simulink model "ForwardKinematic_YuMi"  (R2024a)
(part 18 of 23)

(2579692110316253*sin(q1R))/4503599627370496))/36893488147419103232 + sin(q2R)*((2579692110316253*cos(q1R))/4503599627370496 - (1917820484151683*sin(q1R))/18014398509481984)))/36893488147419103232) + ((234819211581865*cos(q4R))/1152921504606846976 + (9007199067919185*sin(q4R))/9007199254740992)*((129801982932889585091297864435361917839115294955*cos(q1R))/5986310706507378352962293074805895248510699696029696 + (296957971066013582975066703729047659005068212725*cos(q2R))/365375409332725729550921208179070754913983135744 + (174598797980560374072834504815488878557302284405*sin(q1R))/1496577676626844588240573268701473812127674924007424 - (67682029681889335677290557259385*cos(q2R)*((1917820484151683*cos(q1R))/18014398509481984 + (2579692110316253*sin(q1R))/4503599627370496))/332306998946228968225951765070086144 + (9007199067919185*sin(q2R)*((2579692110316253*cos(q1R))/4503599627370496 - (1917820484151683*sin(q1R))/18014398509481984))/9007199254740992 + 206672498930123057048696703425560088887371380901/6129982163463555433433388108601236734474956488734408704)))/36893488147419103232 + sin(q5R)*(((7514214926474921*cos(q4R))/36893488147419103232 + (4503599440548691*sin(q4R))/4503599627370496)*(cos(q3R)*(cos(q2R)*((2579692110316253*cos(q1R))/4503599627370496 - (1917820484151683*sin(q1R))/18014398509481984) - (32968958366167862000829996477285*sin(q2R))/40564819207303340847894502572032 + (7514214926474921*sin(q2R)*((1917820484151683*cos(q1R))/18014398509481984 + (2579692110316253*sin(q1R))/4503599627370496))/36893488147419103232) - (9007199067919185*sin(q3R)*((17274190877287359225804725738355*cos(q1R))/162259276829213363391578010288128 + (23235800371559029388956996013805*sin(q1R))/40564819207303340847894502572032 + 27504203825998033884751021716381/166153499473114484112975882535043072))/9007199254740992 + (7514214926474921*sin(q3R)*((32968958366167862000829996477285*cos(q2R))/40564819207303340847894502572032 - (7514214926474921*cos(q2R)*((1917820484151683*cos(q1R))/18014398509481984 + (2579692110316253*sin(q1R))/4503599627370496))/36893488147419103232 + sin(q2R)*((2579692110316253*cos(q1R))/4503599627370496 - (1917820484151683*sin(q1R))/18014398509481984)))/36893488147419103232) - (7514214926474921*sin(q4R)*((9007199067919185*cos(q3R)*((17274190877287359225804725738355*cos(q1R))/162259276829213363391578010288128 + (23235800371559029388956996013805*sin(q1R))/40564819207303340847894502572032 + 27504203825998033884751021716381/166153499473114484112975882535043072))/9007199254740992 - (7514214926474921*cos(q3R)*((32968958366167862000829996477285*cos(q2R))/40564819207303340847894502572032 - (7514214926474921*cos(q2R)*((1917820484151683*cos(q1R))/18014398509481984 + (2579692110316253*sin(q1R))/4503599627370496))/36893488147419103232 + sin(q2R)*((2579692110316253*cos(q1R))/4503599627370496 - (1917820484151683*sin(q1R))/18014398509481984)))/36893488147419103232 + sin(q3R)*(cos(q2R)*((2579692110316253*cos(q1R))/4503599627370496 - (1917820484151683*sin(q1R))/18014398509481984) - (32968958366167862000829996477285*sin(q2R))/40564819207303340847894502572032 + (7514214926474921*sin(q2R)*((1917820484151683*cos(q1R))/18014398509481984 + (2579692110316253*sin(q1R))/4503599627370496))/36893488147419103232)))/36893488147419103232 + ((9007199067919185*cos(q4R))/9007199254740992 - (234819211581865*sin(q4R))/1152921504606846976)*((129801982932889585091297864435361917839115294955*cos(q1R))/5986310706507378352962293074805895248510699696029696 + (296957971066013582975066703729047659005068212725*cos(q2R))/365375409332725729550921208179070754913983135744 + (174598797980560374072834504815488878557302284405*sin(q1R))/1496577676626844588240573268701473812127674924007424 - (67682029681889335677290557259385*cos(q2R)*((1917820484151683*cos(q1R))/18014398509481984 + (2579692110316253*sin(q1R))/4503599627370496))/332306998946228968225951765070086144 + (9007199067919185*sin(q2R)*((2579692110316253*cos(q1R))/4503599627370496 - (1917820484151683*sin(q1R))/18014398509481984))/9007199254740992 + 206672498930123057048696703425560088887371380901/6129982163463555433433388108601236734474956488734408704))))/9007199254740992000, (584133382113593486367040631332731*sin(q6R)*((1528559695827542654859482295756575375660057523072748460051910118126597762297125*cos(q1R))/8343699359066055009355553539724812947666814540455674882605631280555545803830627148527195652096 + (3497003479222003021661409533057350838749300515155764632398442290070889008826875*cos(q2R))/509258994083621521567111422102344540262867098416484062659035112338595324940834176545849344 + (2056090974134078155817856050893176283501835309672875224633265471054954772650875*sin(q1R))/2085924839766513752338888384931203236916703635113918720651407820138886450957656787131798913024 - (609625514665592237562888769449172969868262801225*cos(q3R)*((17274190877287359225804725738355*cos(q1R))/162259276829213363391578010288128 + (23235800371559029388956996013805*sin(q1R))/40564819207303340847894502572032 + 27504203825998033884751021716381/166153499473114484112975882535043072))/2993155353253689176481146537402947624255349848014848 + (15893040848161638993908057577265778144967053025*sin(q3R)*((17274190877287359225804725738355*cos(q1R))/162259276829213363391578010288128 + (23235800371559029388956996013805*sin(q1R))/40564819207303340847894502572032 + 27504203825998033884751021716381/166153499473114484112975882535043072))/383123885216472214589586756787577295904684780545900544 - (9007199067919185*((4503599440548691*cos(q4R))/4503599627370496 - (7514214926474921*sin(q4R))/36893488147419103232)*(cos(q3R)*(cos(q2R)*((2579692110316253*cos(q1R))/4503599627370496 - (1917820484151683*sin(q1R))/18014398509481984) - (32968958366167862000829996477285*sin(q2R))/40564819207303340847894502572032 + (7514214926474921*sin(q2R)*((1917820484151683*cos(q1R))/18014398509481984 + (2579692110316253*sin(q1R))/4503599627370496))/36893488147419103232) - (9007199067919185*sin(q3R)*((17274190877287359225804725738355*cos(q1R))/162259276829213363391578010288128 + (23235800371559029388956996013805*sin(q1R))/40564819207303340847894502572032 + 27504203825998033884751021716381/166153499473114484112975882535043072))/9007199254740992 + (7514214926474921*sin(q3R)*((32968958366167862000829996477285*cos(q2R))/40564819207303340847894502572032 - (7514214926474921*cos(q2R)*((1917820484151683*cos(q1R))/18014398509481984 + (2579692110316253*sin(q1R))/4503599627370496))/36893488147419103232 + sin(q2R)*((2579692110316253*cos(q1R))/4503599627370496 - (1917820484151683*sin(q1R))/18014398509481984)))/36893488147419103232))/9007199254740992 + (508577317689771495245073589786522929324694383585*cos(q3R)*((32968958366167862000829996477285*cos(q2R))/40564819207303340847894502572032 - (7514214926474921*cos(q2R)*((1917820484151683*cos(q1R))/18014398509481984 + (2579692110316253*sin(q1R))/4503599627370496))/36893488147419103232 + sin(q2R)*((2579692110316253*cos(q1R))/4503599627370496 - (1917820484151683*sin(q1R))/18014398509481984)))/12259964326927110866866776217202473468949912977468817408 - (1764482024691522628700660907665*cos(q3R)*(cos(q2R)*((2579692110316253*cos(q1R))/4503599627370496 - (1917820484151683*sin(q1R))/18014398509481984) - (32968958366167862000829996477285*sin(q2R))/40564819207303340847894502572032 + (7514214926474921*sin(q2R)*((1917820484151683*cos(q1R))/18014398509481984 + (2579692110316253*sin(q1R))/4503599627370496))/36893488147419103232))/42535295865117307932921825928971026432 - (13258697167433729449897784796786197386719169465*sin(q3R)*((32968958366167862000829996477285*cos(q2R))/40564819207303340847894502572032 - (7514214926474921*cos(q2R)*((1917820484151683*cos(q1R))/18014398509481984 + (2579692110316253*sin(q1R))/4503599627370496))/36893488147419103232 + sin(q2R)*((2579692110316253*cos(q1R))/4503599627370496 - (1917820484151683*sin(q1R))/18014398509481984)))/1569275433846670190958947355801916604025588861116008628224 - (67682029681889335677290557259385*sin(q3R)*(cos(q2R)*((2579692110316253*cos(q1R))/4503599627370496 - (1917820484151683*sin(q1R))/18014398509481984) - (32968958366167862000829996477285*sin(q2R))/40564819207303340847894502572032 + (7514214926474921*sin(q2R)*((1917820484151683*cos(q1R))/18014398509481984 + (2579692110316253*sin(q1R))/4503599627370496))/36893488147419103232))/332306998946228968225951765070086144 + (67682029681889335677290557259385*cos(q4R)*((9007199067919185*cos(q3R)*((17274190877287359225804725738355*cos(q1R))/162259276829213363391578010288128 + (23235800371559029388956996013805*sin(q1R))/40564819207303340847894502572032 + 27504203825998033884751021716381/166153499473114484112975882535043072))/9007199254740992 - (7514214926474921*cos(q3R)*((32968958366167862000829996477285*cos(q2R))/40564819207303340847894502572032 - (7514214926474921*cos(q2R)*((1917820484151683*cos(q1R))/18014398509481984 + (2579692110316253*sin(q1R))/4503599627370496))/36893488147419103232 + sin(q2R)*((2579692110316253*cos(q1R))/4503599627370496 - (1917820484151683*sin(q1R))/18014398509481984)))/36893488147419103232 + sin(q3R)*(cos(q2R)*((2579692110316253*cos(q1R))/4503599627370496 - (1917820484151683*sin(q1R))/18014398509481984) - (32968958366167862000829996477285*sin(q2R))/40564819207303340847894502572032 + (7514214926474921*sin(q2R)*((1917820484151683*cos(q1R))/18014398509481984 + (2579692110316253*sin(q1R))/4503599627370496))/36893488147419103232)))/332306998946228968225951765070086144 + (9007199067919185*((234819211581865*cos(q4R))/1152921504606846976 + (9007199067919185*sin(q4R))/9007199254740992)*((129801982932889585091297864435361917839115294955*cos(q1R))/5986310706507378352962293074805895248510699696029696 + (296957971066013582975066703729047659005068212725*cos(q2R))/365375409332725729550921208179070754913983135744 + (174598797980560374072834504815488878557302284405*sin(q1R))/1496577676626844588240573268701473812127674924007424 - (67682029681889335677290557259385*cos(q2R)*((1917820484151683*cos(q1R))/18014398509481984 + (2579692110316253*sin(q1R))/4503599627370496))/332306998946228968225951765070086144 + (9007199067919185*sin(q2R)*((2579692110316253*cos(q1R))/4503599627370496 - (1917820484151683*sin(q1R))/18014398509481984))/9007199254740992 + 206672498930123057048696703425560088887371380901/6129982163463555433433388108601236734474956488734408704))/9007199254740992 - (797029601289130257223357069404502671534492977261568326111352375*cos(q2R)*((1917820484151683*cos(q1R))/18014398509481984 + (2579692110316253*sin(q1R))/4503599627370496))/463168356949264781694283940034751631413079938662562256157830336031652518559744 + (106069577339469832923929692356850887620017617375*sin(q2R)*((2579692110316253*cos(q1R))/4503599627370496 - (1917820484151683*sin(q1R))/18014398509481984))/12554203470773361527671578846415332832204710888928069025792 + 2433793729205816076131138531933890152433695130941136279164373721607455952153675/8543948143683640329580086824678208458410818089426611079788166431288878903122562200091848347746304))/16225927682921336339157801028812800 - (48638874966763599*cos(q6R)*((1528559695827542654859482295756575375660057523072748460051910118126597762297125*cos(q1R))/8343699359066055009355553539724812947666814540455674882605631280555545803830627148527195652096 + (3497003479222003021661409533057350838749300515155764632398442290070889008826875*cos(q2R))/509258994083621521567111422102344540262867098416484062659035112338595324940834176545849344 + (2056090974134078155817856050893176283501835309672875224633265471054954772650875*sin(q1R))/2085924839766513752338888384931203236916703635113918720651407820138886450957656787131798913024 - (609625514665592237562888769449172969868262801225*cos(q3R)*((17274190877287359225804725738355*cos(q1R))/162259276829213363391578010288128 + (23235800371559029388956996013805*sin(q1R))/40564819207303340847894502572032 + 27504203825998033884751021716381/166153499473114484112975882535043072))/2993155353253689176481146537402947624255349848014848 + (15893040848161638993908057577265778144967053025*sin(q3R)*((17274190877287359225804725738355*cos(q1R))/162259276829213363391578010288128 + (23235800371559029388956996013805*sin(q1R))/40564819207303340847894502572032 + 27504203825998033884751021716381/166153499473114484112975882535043072))/383123885216472214589586756787577295904684780545900544 - (9007199067919185*((4503599440548691*cos(q4R))/4503599627370496 - (7514214926474921*sin(q4R))/36893488147419103232)*(cos(q3R)*(cos(q2R)*((2579692110316253*cos(q1R))/4503599627370496 - (1917820484151683*sin(q1R))/18014398509481984) - (32968958366167862000829996477285*sin(q2R))/40564819207303340847894502572032 + (7514214926474921*sin(q2R)*((1917820484151683*cos(q1R))/18014398509481984 + (2579692110316253*sin(q1R))/4503599627370496))/36893488147419103232) - (9007199067919185*sin(q3R)*((17274190877287359225804725738355*cos(q1R))/162259276829213363391578010288128 + (23235800371559029388956996013805*sin(q1R))/40564819207303340847894502572032 + 27504203825998033884751021716381/166153499473114484112975882535043072))/9007199254740992 + (7514214926474921*sin(q3R)*((32968958366167862000829996477285*cos(q2R))/40564819207303340847894502572032 - (7514214926474921*cos(q2R)*((1917820484151683*cos(q1R))/18014398509481984 + (2579692110316253*sin(q1R))/4503599627370496))/36893488147419103232 + sin(q2R)*((2579692110316253*cos(q1R))/4503599627370496 - (1917820484151683*sin(q1R))/18014398509481984)))/36893488147419103232))/9007199254740992 + (508577317689771495245073589786522929324694383585*cos(q3R)*((32968958366167862000829996477285*cos(q2R))/40564819207303340847894502572032 - (7514214926474921*cos(q2R)*((1917820484151683*cos(q1R))/18014398509481984 + (2579692110316253*sin(q1R))/4503599627370496))/36893488147419103232 + sin(q2R)*((2579692110316253*cos(q1R))/4503599627370496 - (1917820484151683*sin(q1R))/18014398509481984)))/12259964326927110866866776217202473468949912977468817408 - (1764482024691522628700660907665*cos(q3R)*(cos(q2R)*((2579692110316253*cos(q1R))/4503599627370496 - (1917820484151683*sin(q1R))/18014398509481984) - (32968958366167862000829996477285*sin(q2R))/40564819207303340847894502572032 + (7514214926474921*sin(q2R)*((1917820484151683*cos(q1R))/18014398509481984 + (2579692110316253*sin(q1R))/4503599627370496))/36893488147419103232))/42535295865117307932921825928971026432 - (13258697167433729449897784796786197386719169465*sin(q3R)*((32968958366167862000829996477285*cos(q2R))/40564819207303340847894502572032 - (7514214926474921*cos(q2R)*((1917820484151683*cos(q1R))/18014398509481984 + (2579692110316253*sin(q1R))/4503599627370496))/36893488147419103232 + sin(q2R)*((2579692110316253*cos(q1R))/4503599627370496 - (1917820484151683*sin(q1R))/18014398509481984)))/1569275433846670190958947355801916604025588861116008628224 - (67682029681889335677290557259385*sin(q3R)*(cos(q2R)*((2579692110316253*cos(q1R))/4503599627370496 - (1917820484151683*sin(q1R))/18014398509481984) - (32968958366167862000829996477285*sin(q2R))/40564819207303340847894502572032 + (7514214926474921*sin(q2R)*((1917820484151683*cos(q1R))/18014398509481984 + (2579692110316253*sin(q1R))/4503599627370496))/36893488147419103232))/332306998946228968225951765070086144 + (67682029681889335677290557259385*cos(q4R)*((9007199067919185*cos(q3R)*((17274190877287359225804725738355*cos(q1R))/162259276829213363391578010288128 + (23235800371559029388956996013805*sin(q1R))/40564819207303340847894502572032 + 27504203825998033884751021716381/166153499473114484112975882535043072))/9007199254740992 - (7514214926474921*cos(q3R)*((32968958366167862000829996477285*cos(q2R))/40564819207303340847894502572032 - (7514214926474921*cos(q2R)*((1917820484151683*cos(q1R))/18014398509481984 + (2579692110316253*sin(q1R))/4503599627370496))/36893488147419103232 + sin(q2R)*((2579692110316253*cos(q1R))/4503599627370496 - (1917820484151683*sin(q1R))/18014398509481984)))/36893488147419103232 + sin(q3R)*(cos(q2R)*((2579692110316253*cos(q1R))/4503599627370496 - (1917820484151683*sin(q1R))/18014398509481984) - (32968958366167862000829996477285*sin(q2R))/40564819207303340847894502572032 + (7514214926474921*sin(q2R)*((1917820484151683*cos(q1R))/18014398509481984 + (2579692110316253*sin(q1R))/4503599627370496))/36893488147419103232)))/332306998946228968225951765070086144 + (9007199067919185*((234819211581865*cos(q4R))/1152921504606846976 + (9007199067919185*sin(q4R))/9007199254740992)*((129801982932889585091297864435361917839115294955*cos(q1R))/5986310706507378352962293074805895248510699696029696 + (296957971066013582975066703729047659005068212725*cos(q2R))/365375409332725729550921208179070754913983135744 + (174598797980560374072834504815488878557302284405*sin(q1R))/1496577676626844588240573268701473812127674924007424 - (67682029681889335677290557259385*cos(q2R)*((1917820484151683*cos(q1R))/18014398509481984 + (2579692110316253*sin(q1R))/4503599627370496))/332306998946228968225951765070086144 + (9007199067919185*sin(q2R)*((2579692110316253*cos(q1R))/4503599627370496 - (1917820484151683*sin(q1R))/18014398509481984))/9007199254740992 + 206672498930123057048696703425560088887371380901/6129982163463555433433388108601236734474956488734408704))/9007199254740992 - (797029601289130257223357069404502671534492977261568326111352375*cos(q2R)*((1917820484151683*cos(q1R))/18014398509481984 + (2579692110316253*sin(q1R))/4503599627370496))/463168356949264781694283940034751631413079938662562256157830336031652518559744 + (106069577339469832923929692356850887620017617375*sin(q2R)*((2579692110316253*cos(q1R))/4503599627370496 - (1917820484151683*sin(q1R))/18014398509481984))/12554203470773361527671578846415332832204710888928069025792 + 2433793729205816076131138531933890152433695130941136279164373721607455952153675/8543948143683640329580086824678208458410818089426611079788166431288878903122562200091848347746304))/1801439850948198400 - (27*sin(q6R)*(cos(q5R)*(((7514214926474921*cos(q4R))/36893488147419103232 + (4503599440548691*sin(q4R))/4503599627370496)*(cos(q3R)*(cos(q2R)*((2579692110316253*cos(q1R))/4503599627370496 - (1917820484151683*sin(q1R))/18014398509481984) - (32968958366167862000829996477285*sin(q2R))/40564819207303340847894502572032 + (7514214926474921*sin(q2R)*((1917820484151683*cos(q1R))/18014398509481984 + (2579692110316253*sin(q1R))/4503599627370496))/36893488147419103232) - (9007199067919185*sin(q3R)*((17274190877287359225804725738355*cos(q1R))/162259276829213363391578010288128 + (23235800371559029388956996013805*sin(q1R))/40564819207303340847894502572032 + 27504203825998033884751021716381/166153499473114484112975882535043072))/9007199254740992 + (7514214926474921*sin(q3R)*((32968958366167862000829996477285*cos(q2R))/40564819207303340847894502572032 - (7514214926474921*cos(q2R)*((1917820484151683*cos(q1R))/18014398509481984 + (2579692110316253*sin(q1R))/4503599627370496))/36893488147419103232 + sin(q2R)*((2579692110316253*cos(q1R))/4503599627370496 - (1917820484151683*sin(q1R))/18014398509481984)))/36893488147419103232) - (7514214926474921*sin(q4R)*((9007199067919185*cos(q3R)*((17274190877287359225804725738355*cos(q1R))/162259276829213363391578010288128 + (23235800371559029388956996013805*sin(q1R))/40564819207303340847894502572032 + 27504203825998033884751021716381/166153499473114484112975882535043072))/9007199254740992 - (7514214926474921*cos(q3R)*((32968958366167862000829996477285*cos(q2R))/40564819207303340847894502572032 - (7514214926474921*cos(q2R)*((1917820484151683*cos(q1R))/18014398509481984 + (2579692110316253*sin(q1R))/4503599627370496))/36893488147419103232 + sin(q2R)*((2579692110316253*cos(q1R))/4503599627370496 - (1917820484151683*sin(q1R))/18014398509481984)))/36893488147419103232 + sin(q3R)*(cos(q2R)*((2579692110316253*cos(q1R))/4503599627370496 - (1917820484151683*sin(q1R))/18014398509481984) - (32968958366167862000829996477285*sin(q2R))/40564819207303340847894502572032 + (7514214926474921*sin(q2R)*((1917820484151683*cos(q1R))/18014398509481984 + (2579692110316253*sin(q1R))/4503599627370496))/36893488147419103232)))/36893488147419103232 + ((9007199067919185*cos(q4R))/9007199254740992 - (234819211581865*sin(q4R))/1152921504606846976)*((129801982932889585091297864435361917839115294955*cos(q1R))/5986310706507378352962293074805895248510699696029696 + (296957971066013582975066703729047659005068212725*cos(q2R))/365375409332725729550921208179070754913983135744 + (174598797980560374072834504815488878557302284405*sin(q1R))/1496577676626844588240573268701473812127674924007424 - (67682029681889335677290557259385*cos(q2R)*((1917820484151683*cos(q1R))/18014398509481984 + (2579692110316253*sin(q1R))/4503599627370496))/332306998946228968225951765070086144 + (9007199067919185*sin(q2R)*((2579692110316253*cos(q1R))/4503599627370496 - (1917820484151683*sin(q1R))/18014398509481984))/9007199254740992 + 206672498930123057048696703425560088887371380901/6129982163463555433433388108601236734474956488734408704)) - (9007199067919185*sin(q5R)*((203422408166946418981152780445187297537016008229516441756292125*cos(q1R))/226156424291633194186662080095093570025917938800079226639565593765455331328 + (465385075279251052437186083221547446448384963368966483726351875*cos(q2R))/13803492693581127574869511724554050904902217944340773110325048447598592 + (273626851807209941619219010639387076236787289365779842797695875*sin(q1R))/56539106072908298546665520023773392506479484700019806659891398441363832832 - (81129635049124235038645691064225*cos(q3R)*((17274190877287359225804725738355*cos(q1R))/162259276829213363391578010288128 + (23235800371559029388956996013805*sin(q1R))/40564819207303340847894502572032 + 27504203825998033884751021716381/166153499473114484112975882535043072))/81129638414606681695789005144064 + (2115063383689692319117831580025*sin(q3R)*((17274190877287359225804725738355*cos(q1R))/162259276829213363391578010288128 + (23235800371559029388956996013805*sin(q1R))/40564819207303340847894502572032 + 27504203825998033884751021716381/166153499473114484112975882535043072))/10384593717069655257060992658440192 + (67682029681889335677290557259385*cos(q3R)*((32968958366167862000829996477285*cos(q2R))/40564819207303340847894502572032 - (7514214926474921*cos(q2R)*((1917820484151683*cos(q1R))/18014398509481984 + (2579692110316253*sin(q1R))/4503599627370496))/36893488147419103232 + sin(q2R)*((2579692110316253*cos(q1R))/4503599627370496 - (1917820484151683*sin(q1R))/18014398509481984)))/332306998946228968225951765070086144 - (234819211581865*cos(q3R)*(cos(q2R)*((2579692110316253*cos(q1R))/4503599627370496 - (1917820484151683*sin(q1R))/18014398509481984) - (32968958366167862000829996477285*sin(q2R))/40564819207303340847894502572032 + (7514214926474921*sin(q2R)*((1917820484151683*cos(q1R))/18014398509481984 + (2579692110316253*sin(q1R))/4503599627370496))/36893488147419103232))/1152921504606846976 - (1764482024691522628700660907665*sin(q3R)*((32968958366167862000829996477285*cos(q2R))/40564819207303340847894502572032 - (7514214926474921*cos(q2R)*((1917820484151683*cos(q1R))/18014398509481984 + (2579692110316253*sin(q1R))/4503599627370496))/36893488147419103232 + sin(q2R)*((2579692110316253*cos(q1R))/4503599627370496 - (1917820484151683*sin(q1R))/18014398509481984)))/42535295865117307932921825928971026432 - (9007199067919185*sin(q3R)*(cos(q2R)*((2579692110316253*cos(q1R))/4503599627370496 - (1917820484151683*sin(q1R))/18014398509481984) - (32968958366167862000829996477285*sin(q2R))/40564819207303340847894502572032 + (7514214926474921*sin(q2R)*((1917820484151683*cos(q1R))/18014398509481984 + (2579692110316253*sin(q1R))/4503599627370496))/36893488147419103232))/9007199254740992 - (106069577339469832923929692356850887620017617375*cos(q2R)*((1917820484151683*cos(q1R))/18014398509481984 + (2579692110316253*sin(q1R))/4503599627370496))/12554203470773361527671578846415332832204710888928069025792 + (14115856197532180673579726082375*sin(q2R)*((2579692110316253*cos(q1R))/4503599627370496 - (1917820484151683*sin(q1R))/18014398509481984))/340282366920938463463374607431768211456 + 323891950525769801103968238055131782751500431270071838086942675/231584178474632390847141970017375815706539969331281128078915168015826259279872))/9007199254740992 + (7514214926474921*sin(q5R)*((7514214926474921*cos(q4R)*((9007199067919185*cos(q3R)*((17274190877287359225804725738355*cos(q1R))/162259276829213363391578010288128 + (23235800371559029388956996013805*sin(q1R))/40564819207303340847894502572032 + 27504203825998033884751021716381/166153499473114484112975882535043072))/9007199254740992 - (7514214926474921*cos(q3R)*((32968958366167862000829996477285*cos(q2R))/40564819207303340847894502572032 - (7514214926474921*cos(q2R)*((1917820484151683*cos(q1R))/18014398509481984 + (2579692110316253*sin(q1R))/4503599627370496))/36893488147419103232 + sin(q2R)*((2579692110316253*cos(q1R))/4503599627370496 - (1917820484151683*sin(q1R))/18014398509481984)))/36893488147419103232 + sin(q3R)*(cos(q2R)*((2579692110316253*cos(q1R))/4503599627370496 - (1917820484151683*sin(q1R))/18014398509481984) - (32968958366167862000829996477285*sin(q2R))/40564819207303340847894502572032 + (7514214926474921*sin(q2R)*((1917820484151683*cos(q1R))/18014398509481984 + (2579692110316253*sin(q1R))/4503599627370496))/36893488147419103232)))/36893488147419103232 - ((4503599440548691*cos(q4R))/4503599627370496 - (7514214926474921*sin(q4R))/36893488147419103232)*(cos(q3R)*(cos(q2R)*((2579692110316253*cos(q1R))/4503599627370496 - (1917820484151683*sin(q1R))/18014398509481984) - (32968958366167862000829996477285*sin(q2R))/40564819207303340847894502572032 + (7514214926474921*sin(q2R)*((1917820484151683*cos(q1R))/18014398509481984 + (2579692110316253*sin(q1R))/4503599627370496))/36893488147419103232) - (9007199067919185*sin(q3R)*((17274190877287359225804725738355*cos(q1R))/162259276829213363391578010288128 + (23235800371559029388956996013805*sin(q1R))/40564819207303340847894502572032 + 27504203825998033884751021716381/166153499473114484112975882535043072))/9007199254740992 + (7514214926474921*sin(q3R)*((32968958366167862000829996477285*cos(q2R))/40564819207303340847894502572032 - (7514214926474921*cos(q2R)*((1917820484151683*cos(q1R))/18014398509481984 + (2579692110316253*sin(q1R))/4503599627370496))/36893488147419103232 + sin(q2R)*((2579692110316253*cos(q1R))/4503599627370496 - (1917820484151683*sin(q1R))/18014398509481984)))/36893488147419103232) + ((234819211581865*cos(q4R))/1152921504606846976 + (9007199067919185*sin(q4R))/9007199254740992)*((129801982932889585091297864435361917839115294955*cos(q1R))/5986310706507378352962293074805895248510699696029696 + (296957971066013582975066703729047659005068212725*cos(q2R))/365375409332725729550921208179070754913983135744 + (174598797980560374072834504815488878557302284405*sin(q1R))/1496577676626844588240573268701473812127674924007424 - (67682029681889335677290557259385*cos(q2R)*((1917820484151683*cos(q1R))/18014398509481984 + (2579692110316253*sin(q1R))/4503599627370496))/332306998946228968225951765070086144 + (9007199067919185*sin(q2R)*((2579692110316253*cos(q1R))/4503599627370496 - (1917820484151683*sin(q1R))/18014398509481984))/9007199254740992 + 206672498930123057048696703425560088887371380901/6129982163463555433433388108601236734474956488734408704)))/36893488147419103232))/1000 + (202883803014822867*cos(q6R)*((9007199067919185*cos(q5R)*((203422408166946418981152780445187297537016008229516441756292125*cos(q1R))/226156424291633194186662080095093570025917938800079226639565593765455331328 + (465385075279251052437186083221547446448384963368966483726351875*cos(q2R))/13803492693581127574869511724554050904902217944340773110325048447598592 + (273626851807209941619219010639387076236787289365779842797695875*sin(q1R))/56539106072908298546665520023773392506479484700019806659891398441363832832 - (81129635049124235038645691064225*cos(q3R)*((17274190877287359225804725738355*cos(q1R))/162259276829213363391578010288128 + (23235800371559029388956996013805*sin(q1R))/40564819207303340847894502572032 + 27504203825998033884751021716381/166153499473114484112975882535043072))/81129638414606681695789005144064 + (2115063383689692319117831580025*sin(q3R)*((17274190877287359225804725738355*cos(q1R))/162259276829213363391578010288128 + (23235800371559029388956996013805*sin(q1R))/40564819207303340847894502572032 + 27504203825998033884751021716381/166153499473114484112975882535043072))/10384593717069655257060992658440192 + (67682029681889335677290557259385*cos(q3R)*((32968958366167862000829996477285*cos(q2R))/40564819207303340847894502572032 - (7514214926474921*cos(q2R)*((1917820484151683*cos(q1R))/18014398509481984 + (2579692110316253*sin(q1R))/4503599627370496))/36893488147419103232 + sin(q2R)*((2579692110316253*cos(q1R))/4503599627370496 - (1917820484151683*sin(q1R))/18014398509481984)))/332306998946228968225951765070086144 - (234819211581865*cos(q3R)*(cos(q2R)*((2579692110316253*cos(q1R))/4503599627370496 - (1917820484151683*sin(q1R))/18014398509481984) - (32968958366167862000829996477285*sin(q2R))/40564819207303340847894502572032 + (7514214926474921*sin(q2R)*((1917820484151683*cos(q1R))/18014398509481984 + (2579692110316253*sin(q1R))/4503599627370496))/36893488147419103232))/1152921504606846976 - (1764482024691522628700660907665*sin(q3R)*((32968958366167862000829996477285*cos(q2R))/40564819207303340847894502572032 - (7514214926474921*cos(q2R)*((1917820484151683*cos(q1R))/18014398509481984 + (2579692110316253*sin(q1R))/4503599627370496))/36893488147419103232 + sin(q2R)*((2579692110316253*cos(q1R))/4503599627370496 - (1917820484151683*sin(q1R))/18014398509481984)))/42535295865117307932921825928971026432 - (9007199067919185*sin(q3R)*(cos(q2R)*((2579692110316253*cos(q1R))/4503599627370496 - (1917820484151683*sin(q1R))/18014398509481984) - (32968958366167862000829996477285*sin(q2R))/40564819207303340847894502572032 + (7514214926474921*sin(q2R)*((1917820484151683*cos(q1R))/18014398509481984 + (2579692110316253*sin(q1R))/4503599627370496))/36893488147419103232))/9007199254740992 - (106069577339469832923929692356850887620017617375*cos(q2R)*((1917820484151683*cos(q1R))/18014398509481984 + (2579692110316253*sin(q1R))/4503599627370496))/12554203470773361527671578846415332832204710888928069025792 + (14115856197532180673579726082375*sin(q2R)*((2579692110316253*cos(q1R))/4503599627370496 - (1917820484151683*sin(q1R))/18014398509481984))/340282366920938463463374607431768211456 + 323891950525769801103968238055131782751500431270071838086942675/231584178474632390847141970017375815706539969331281128078915168015826259279872))/9007199254740992 - (7514214926474921*cos(q5R)*((7514214926474921*cos(q4R)*((9007199067919185*cos(q3R)*((17274190877287359225804725738355*cos(q1R))/162259276829213363391578010288128 + (23235800371559029388956996013805*sin(q1R))/40564819207303340847894502572032 + 27504203825998033884751021716381/166153499473114484112975882535043072))/9007199254740992 - (7514214926474921*cos(q3R)*((32968958366167862000829996477285*cos(q2R))/40564819207303340847894502572032 - (7514214926474921*cos(q2R)*((1917820484151683*cos(q1R))/18014398509481984 + (2579692110316253*sin(q1R))/4503599627370496))/36893488147419103232 + sin(q2R)*((2579692110316253*cos(q1R))/4503599627370496 - (1917820484151683*sin(q1R))/18014398509481984)))/36893488147419103232 + sin(q3R)*(cos(q2R)*((2579692110316253*cos(q1R))/4503599627370496 - (1917820484151683*sin(q1R))/18014398509481984) - (32968958366167862000829996477285*sin(q2R))/40564819207303340847894502572032 + (7514214926474921*sin(q2R)*((1917820484151683*cos(q1R))/18014398509481984 + (2579692110316253*sin(q1R))/4503599627370496))/36893488147419103232)))/36893488147419103232 - ((4503599440548691*cos(q4R))/4503599627370496 - (7514214926474921*sin(q4R))/36893488147419103232)*(cos(q3R)*(cos(q2R)*((2579692110316253*cos(q1R))/4503599627370496 - (1917820484151683*sin(q1R))/18014398509481984) - (32968958366167862000829996477285*sin(q2R))/40564819207303340847894502572032 + (7514214926474921*sin(q2R)*((1917820484151683*cos(q1R))/18014398509481984 + (2579692110316253*sin(q1R))/4503599627370496))/36893488147419103232) - (9007199067919185*sin(q3R)*((17274190877287359225804725738355*cos(q1R))/162259276829213363391578010288128 + (23235800371559029388956996013805*sin(q1R))/40564819207303340847894502572032 + 27504203825998033884751021716381/166153499473114484112975882535043072))/9007199254740992 + (7514214926474921*sin(q3R)*((32968958366167862000829996477285*cos(q2R))/40564819207303340847894502572032 - (7514214926474921*cos(q2R)*((1917820484151683*cos(q1R))/18014398509481984 + (2579692110316253*sin(q1R))/4503599627370496))/36893488147419103232 + sin(q2R)*((2579692110316253*cos(q1R))/4503599627370496 - (1917820484151683*sin(q1R))/18014398509481984)))/36893488147419103232) + ((234819211581865*cos(q4R))/1152921504606846976 + (9007199067919185*sin(q4R))/9007199254740992)*((129801982932889585091297864435361917839115294955*cos(q1R))/5986310706507378352962293074805895248510699696029696 + (296957971066013582975066703729047659005068212725*cos(q2R))/365375409332725729550921208179070754913983135744 + (174598797980560374072834504815488878557302284405*sin(q1R))/1496577676626844588240573268701473812127674924007424 - (67682029681889335677290557259385*cos(q2R)*((1917820484151683*cos(q1R))/18014398509481984 + (2579692110316253*sin(q1R))/4503599627370496))/332306998946228968225951765070086144 + (9007199067919185*sin(q2R)*((2579692110316253*cos(q1R))/4503599627370496 - (1917820484151683*sin(q1R))/18014398509481984))/9007199254740992 + 206672498930123057048696703425560088887371380901/6129982163463555433433388108601236734474956488734408704)))/36893488147419103232 + sin(q5R)*(((7514214926474921*cos(q4R))/36893488147419103232 + (4503599440548691*sin(q4R))/4503599627370496)*(cos(q3R)*(cos(q2R)*((2579692110316253*cos(q1R))/4503599627370496 - (1917820484151683*sin(q1R))/18014398509481984) - (32968958366167862000829996477285*sin(q2R))/40564819207303340847894502572032 + (7514214926474921*sin(q2R)*((1917820484151683*cos(q1R))/18014398509481984 + (2579692110316253*sin(q1R))/4503599627370496))/36893488147419103232) - (9007199067919185*sin(q3R)*((17274190877287359225804725738355*cos(q1R))/162259276829213363391578010288128 + (23235800371559029388956996013805*sin(q1R))/40564819207303340847894502572032 + 27504203825998033884751021716381/166153499473114484112975882535043072))/9007199254740992 + (7514214926474921*sin(q3R)*((32968958366167862000829996477285*cos(q2R))/40564819207303340847894502572032 - (7514214926474921*cos(q2R)*((1917820484151683*cos(q1R))/18014398509481984 + (2579692110316253*sin(q1R))/4503599627370496))/36893488147419103232 + sin(q2R)*((2579692110316253*cos(q1R))/4503599627370496 - (1917820484151683*sin(q1R))/18014398509481984)))/36893488147419103232) - (7514214926474921*sin(q4R)*((9007199067919185*cos(q3R)*((17274190877287359225804725738355*cos(q1R))/162259276829213363391578010288128 + (23235800371559029388956996013805*sin(q1R))/40564819207303340847894502572032 + 27504203825998033884751021716381/166153499473114484112975882535043072))/9007199254740992 - (7514214926474921*cos(q3R)*((32968958366167862000829996477285*cos(q2R))/40564819207303340847894502572032 - (7514214926474921*cos(q2R)*((1917820484151683*cos(q1R))/18014398509481984 + (2579692110316253*sin(q1R))/4503599627370496))/36893488147419103232 + sin(q2R)*((2579692110316253*cos(q1R))/4503599627370496 - (1917820484151683*sin(q1R))/18014398509481984)))/36893488147419103232 + sin(q3R)*(cos(q2R)*((2579692110316253*cos(q1R))/4503599627370496 - (1917820484151683*sin(q1R))/18014398509481984) - (32968958366167862000829996477285*sin(q2R))/40564819207303340847894502572032 + (7514214926474921*sin(q2R)*((1917820484151683*cos(q1R))/18014398509481984 + (2579692110316253*sin(q1R))/4503599627370496))/36893488147419103232)))/36893488147419103232 + ((9007199067919185*cos(q4R))/9007199254740992 - (234819211581865*sin(q4R))/1152921504606846976)*((129801982932889585091297864435361917839115294955*cos(q1R))/5986310706507378352962293074805895248510699696029696 + (296957971066013582975066703729047659005068212725*cos(q2R))/365375409332725729550921208179070754913983135744 + (174598797980560374072834504815488878557302284405*sin(q1R))/1496577676626844588240573268701473812127674924007424 - (67682029681889335677290557259385*cos(q2R)*((1917820484151683*cos(q1R))/18014398509481984 + (2579692110316253*sin(q1R))/4503599627370496))/332306998946228968225951765070086144 + (9007199067919185*sin(q2R)*((2579692110316253*cos(q1R))/4503599627370496 - (1917820484151683*sin(q1R))/18014398509481984))/9007199254740992 + 206672498930123057048696703425560088887371380901/6129982163463555433433388108601236734474956488734408704))))/36893488147419103232000 - (324259171862923063*cos(q6R)*(cos(q5R)*(((7514214926474921*cos(q4R))/36893488147419103232 + (4503599440548691*sin(q4R))/4503599627370496)*(cos(q3R)*(cos(q2R)*((2579692110316253*cos(q1R))/4503599627370496 - (1917820484151683*sin(q1R))/18014398509481984) - (32968958366167862000829996477285*sin(q2R))/40564819207303340847894502572032 + (7514214926474921*sin(q2R)*((1917820484151683*cos(q1R))/18014398509481984 + (2579692110316253*sin(q1R))/4503599627370496))/36893488147419103232) - (9007199067919185*sin(q3R)*((17274190877287359225804725738355*cos(q1R))/162259276829213363391578010288128 + (23235800371559029388956996013805*sin(q1R))/40564819207303340847894502572032 + 27504203825998033884751021716381/166153499473114484112975882535043072))/9007199254740992 + (7514214926474921*sin(q3R)*((32968958366167862000829996477285*cos(q2R))/40564819207303340847894502572032 - (7514214926474921*cos(q2R)*((1917820484151683*cos(q1R))/18014398509481984 + (2579692110316253*sin(q1R))/4503599627370496))/36893488147419103232 + sin(q2R)*((2579692110316253*cos(q1R))/4503599627370496 - (1917820484151683*sin(q1R))/18014398509481984)))/36893488147419103232) - (7514214926474921*sin(q4R)*((9007199067919185*cos(q3R)*((17274190877287359225804725738355*cos(q1R))/162259276829213363391578010288128 + (23235800371559029388956996013805*sin(q1R))/40564819207303340847894502572032 + 27504203825998033884751021716381/166153499473114484112975882535043072))/9007199254740992 - (7514214926474921*cos(q3R)*((32968958366167862000829996477285*cos(q2R))/40564819207303340847894502572032 - (7514214926474921*cos(q2R)*((1917820484151683*cos(q1R))/18014398509481984 + (2579692110316253*sin(q1R))/4503599627370496))/36893488147419103232 + sin(q2R)*((2579692110316253*cos(q1R))/4503599627370496 - (1917820484151683*sin(q1R))/18014398509481984)))/36893488147419103232 + sin(q3R)*(cos(q2R)*((2579692110316253*cos(q1R))/4503599627370496 - (1917820484151683*sin(q1R))/18014398509481984) - (32968958366167862000829996477285*sin(q2R))/40564819207303340847894502572032 + (7514214926474921*sin(q2R)*((1917820484151683*cos(q1R))/18014398509481984 + (2579692110316253*sin(q1R))/4503599627370496))/36893488147419103232)))/36893488147419103232 + ((9007199067919185*cos(q4R))/9007199254740992 - (234819211581865*sin(q4R))/1152921504606846976)*((129801982932889585091297864435361917839115294955*cos(q1R))/5986310706507378352962293074805895248510699696029696 + (296957971066013582975066703729047659005068212725*cos(q2R))/365375409332725729550921208179070754913983135744 + (174598797980560374072834504815488878557302284405*sin(q1R))/1496577676626844588240573268701473812127674924007424 - (67682029681889335677290557259385*cos(q2R)*((1917820484151683*cos(q1R))/18014398509481984 + (2579692110316253*sin(q1R))/4503599627370496))/332306998946228968225951765070086144 + (9007199067919185*sin(q2R)*((2579692110316253*cos(q1R))/4503599627370496 - (1917820484151683*sin(q1R))/18014398509481984))/9007199254740992 + 206672498930123057048696703425560088887371380901/6129982163463555433433388108601236734474956488734408704)) - (9007199067919185*sin(q5R)*((203422408166946418981152780445187297537016008229516441756292125*cos(q1R))/226156424291633194186662080095093570025917938800079226639565593765455331328 + (465385075279251052437186083221547446448384963368966483726351875*cos(q2R))/13803492693581127574869511724554050904902217944340773110325048447598592 + (273626851807209941619219010639387076236787289365779842797695875*sin(q1R))/56539106072908298546665520023773392506479484700019806659891398441363832832 - (81129635049124235038645691064225*cos(q3R)*((17274190877287359225804725738355*cos(q1R))/162259276829213363391578010288128 + (23235800371559029388956996013805*sin(q1R))/40564819207303340847894502572032 + 27504203825998033884751021716381/166153499473114484112975882535043072))/81129638414606681695789005144064 + (2115063383689692319117831580025*sin(q3R)*((17274190877287359225804725738355*cos(q1R))/162259276829213363391578010288128 + (23235800371559029388956996013805*sin(q1R))/40564819207303340847894502572032 + 27504203825998033884751021716381/166153499473114484112975882535043072))/10384593717069655257060992658440192 + (67682029681889335677290557259385*cos(q3R)*((32968958366167862000829996477285*cos(q2R))/40564819207303340847894502572032 - (7514214926474921*cos(q2R)*((1917820484151683*cos(q1R))/18014398509481984 + (2579692110316253*sin(q1R))/4503599627370496))/36893488147419103232 + sin(q2R)*((2579692110316253*cos(q1R))/4503599627370496 - (1917820484151683*sin(q1R))/18014398509481984)))/332306998946228968225951765070086144 - (234819211581865*cos(q3R)*(cos(q2R)*((2579692110316253*cos(q1R))/4503599627370496 - (1917820484151683*sin(q1R))/18014398509481984) - (32968958366167862000829996477285*sin(q2R))/40564819207303340847894502572032 + (7514214926474921*sin(q2R)*((1917820484151683*cos(q1R))/18014398509481984 + (2579692110316253*sin(q1R))/4503599627370496))/36893488147419103232))/1152921504606846976 - (1764482024691522628700660907665*sin(q3R)*((32968958366167862000829996477285*cos(q2R))/40564819207303340847894502572032 - (7514214926474921*cos(q2R)*((1917820484151683*cos(q1R))/18014398509481984 + (2579692110316253*sin(q1R))/4503599627370496))/36893488147419103232 + sin(q2R)*((2579692110316253*cos(q1R))/4503599627370496 - (1917820484151683*sin(q1R))/18014398509481984)))/42535295865117307932921825928971026432 - (9007199067919185*sin(q3R)*(cos(q2R)*((2579692110316253*cos(q1R))/4503599627370496 - (1917820484151683*sin(q1R))/18014398509481984) - (32968958366167862000829996477285*sin(q2R))/40564819207303340847894502572032 + (7514214926474921*sin(q2R)*((1917820484151683*cos(q1R))/18014398509481984 + (2579692110316253*sin(q1R))/4503599627370496))/36893488147419103232))/9007199254740992 - (106069577339469832923929692356850887620017617375*cos(q2R)*((1917820484151683*cos(q1R))/18014398509481984 + (2579692110316253*sin(q1R))/4503599627370496))/12554203470773361527671578846415332832204710888928069025792 + (14115856197532180673579726082375*sin(q2R)*((2579692110316253*cos(q1R))/4503599627370496 - (1917820484151683*sin(q1R))/18014398509481984))/340282366920938463463374607431768211456 + 323891950525769801103968238055131782751500431270071838086942675/231584178474632390847141970017375815706539969331281128078915168015826259279872))/9007199254740992 + (7514214926474921*sin(q5R)*((7514214926474921*cos(q4R)*((9007199067919185*cos(q3R)*((17274190877287359225804725738355*cos(q1R))/162259276829213363391578010288128 + (23235800371559029388956996013805*sin(q1R))/40564819207303340847894502572032 + 27504203825998033884751021716381/166153499473114484112975882535043072))/9007199254740992 - (7514214926474921*cos(q3R)*((32968958366167862000829996477285*cos(q2R))/40564819207303340847894502572032 - (7514214926474921*cos(q2R)*((1917820484151683*cos(q1R))/18014398509481984 + (2579692110316253*sin(q1R))/4503599627370496))/36893488147419103232 + sin(q2R)*((2579692110316253*cos(q1R))/4503599627370496 - (1917820484151683*sin(q1R))/18014398509481984)))/36893488147419103232 + sin(q3R)*(cos(q2R)*((2579692110316253*cos(q1R))/4503599627370496 - (1917820484151683*sin(q1R))/18014398509481984) - (32968958366167862000829996477285*sin(q2R))/40564819207303340847894502572032 + (7514214926474921*sin(q2R)*((1917820484151683*cos(q1R))/18014398509481984 + (2579692110316253*sin(q1R))/4503599627370496))/36893488147419103232)))/36893488147419103232 - ((4503599440548691*cos(q4R))/4503599627370496 - (7514214926474921*sin(q4R))/36893488147419103232)*(cos(q3R)*(cos(q2R)*((2579692110316253*cos(q1R))/4503599627370496 - (1917820484151683*sin(q1R))/18014398509481984) - (32968958366167862000829996477285*sin(q2R))/40564819207303340847894502572032 + (7514214926474921*sin(q2R)*((1917820484151683*cos(q1R))/18014398509481984 + (2579692110316253*sin(q1R))/4503599627370496))/36893488147419103232) - (9007199067919185*sin(q3R)*((17274190877287359225804725738355*cos(q1R))/162259276829213363391578010288128 + (23235800371559029388956996013805*sin(q1R))/40564819207303340847894502572032 + 27504203825998033884751021716381/166153499473114484112975882535043072))/9007199254740992 + (7514214926474921*sin(q3R)*((32968958366167862000829996477285*cos(q2R))/40564819207303340847894502572032 - (7514214926474921*cos(q2R)*((1917820484151683*cos(q1R))/18014398509481984 + (2579692110316253*sin(q1R))/4503599627370496))/36893488147419103232 + sin(q2R)*((2579692110316253*cos(q1R))/4503599627370496 - (1917820484151683*sin(q1R))/18014398509481984)))/36893488147419103232) + ((234819211581865*cos(q4R))/1152921504606846976 + (9007199067919185*sin(q4R))/9007199254740992)*((129801982932889585091297864435361917839115294955*cos(q1R))/5986310706507378352962293074805895248510699696029696 + (296957971066013582975066703729047659005068212725*cos(q2R))/365375409332725729550921208179070754913983135744 + (174598797980560374072834504815488878557302284405*sin(q1R))/1496577676626844588240573268701473812127674924007424 - (67682029681889335677290557259385*cos(q2R)*((1917820484151683*cos(q1R))/18014398509481984 + (2579692110316253*sin(q1R))/4503599627370496))/332306998946228968225951765070086144 + (9007199067919185*sin(q2R)*((2579692110316253*cos(q1R))/4503599627370496 - (1917820484151683*sin(q1R))/18014398509481984))/9007199254740992 + 206672498930123057048696703425560088887371380901/6129982163463555433433388108601236734474956488734408704)))/36893488147419103232))/9007199254740992000 - (2436553109258773196144549622003023*sin(q6R)*((9007199067919185*cos(q5R)*((203422408166946418981152780445187297537016008229516441756292125*cos(q1R))/226156424291633194186662080095093570025917938800079226639565593765455331328 + (465385075279251052437186083221547446448384963368966483726351875*cos(q2R))/13803492693581127574869511724554050904902217944340773110325048447598592 + (273626851807209941619219010639387076236787289365779842797695875*sin(q1R))/56539106072908298546665520023773392506479484700019806659891398441363832832 - (81129635049124235038645691064225*cos(q3R)*((17274190877287359225804725738355*cos(q1R))/162259276829213363391578010288128 + (23235800371559029388956996013805*sin(q1R))/40564819207303340847894502572032 + 27504203825998033884751021716381/166153499473114484112975882535043072))/81129638414606681695789005144064 + (2115063383689692319117831580025*sin(q3R)*((17274190877287359225804725738355*cos(q1R))/162259276829213363391578010288128 + (23235800371559029388956996013805*sin(q1R))/40564819207303340847894502572032 + 27504203825998033884751021716381/166153499473114484112975882535043072))/10384593717069655257060992658440192 + (67682029681889335677290557259385*cos(q3R)*((32968958366167862000829996477285*cos(q2R))/40564819207303340847894502572032 - (7514214926474921*cos(q2R)*((1917820484151683*cos(q1R))/18014398509481984 + (2579692110316253*sin(q1R))/4503599627370496))/36893488147419103232 + sin(q2R)*((2579692110316253*cos(q1R))/4503599627370496 - (1917820484151683*sin(q1R))/18014398509481984)))/332306998946228968225951765070086144 - (234819211581865*cos(q3R)*(cos(q2R)*((2579692110316253*cos(q1R))/4503599627370496 - (1917820484151683*sin(q1R))/18014398509481984) - (32968958366167862000829996477285*sin(q2R))/40564819207303340847894502572032 + (7514214926474921*sin(q2R)*((1917820484151683*cos(q1R))/18014398509481984 + (2579692110316253*sin(q1R))/4503599627370496))/36893488147419103232))/1152921504606846976 - (1764482024691522628700660907665*sin(q3R)*((32968958366167862000829996477285*cos(q2R))/40564819207303340847894502572032 - (7514214926474921*cos(q2R)*((1917820484151683*cos(q1R))/18014398509481984 + (2579692110316253*sin(q1R))/4503599627370496))/36893488147419103232 + sin(q2R)*((2579692110316253*cos(q1R))/4503599627370496 - (1917820484151683*sin(q1R))/18014398509481984)))/42535295865117307932921825928971026432 - (9007199067919185*sin(q3R)*(cos(q2R)*((2579692110316253*cos(q1R))/4503599627370496 - (1917820484151683*sin(q1R))/18014398509481984) - (32968958366167862000829996477285*sin(q2R))/40564819207303340847894502572032 + (7514214926474921*sin(q2R)*((1917820484151683*cos(q1R))/18014398509481984 + (2579692110316253*sin(q1R))/4503599627370496))/36893488147419103232))/9007199254740992 - (106069577339469832923929692356850887620017617375*cos(q2R)*((1917820484151683*cos(q1R))/18014398509481984 + (2579692110316253*sin(q1R))/4503599627370496))/12554203470773361527671578846415332832204710888928069025792 + (14115856197532180673579726082375*sin(q2R)*((2579692110316253*cos(q1R))/4503599627370496 - (1917820484151683*sin(q1R))/18014398509481984))/340282366920938463463374607431768211456 + 323891950525769801103968238055131782751500431270071838086942675/231584178474632390847141970017375815706539969331281128078915168015826259279872))/9007199254740992 - (7514214926474921*cos(q5R)*((7514214926474921*cos(q4R)*((9007199067919185*cos(q3R)*((17274190877287359225804725738355*cos(q1R))/162259276829213363391578010288128 + (23235800371559029388956996013805*sin(q1R))/40564819207303340847894502572032 + 27504203825998033884751021716381/166153499473114484112975882535043072))/9007199254740992 - (7514214926474921*cos(q3R)*((32968958366167862000829996477285*cos(q2R))/40564819207303340847894502572032 - (7514214926474921*cos(q2R)*((1917820484151683*cos(q1R))/18014398509481984 + (2579692110316253*sin(q1R))/4503599627370496))/36893488147419103232 + sin(q2R)*((2579692110316253*cos(q1R))/4503599627370496 - (1917820484151683*sin(q1R))/18014398509481984)))/36893488147419103232 + sin(q3R)*(cos(q2R)*((2579692110316253*cos(q1R))/4503599627370496 - (1917820484151683*sin(q1R))/18014398509481984) - (32968958366167862000829996477285*sin(q2R))/40564819207303340847894502572032 + (7514214926474921*sin(q2R)*((1917820484151683*cos(q1R))/18014398509481984 + (2579692110316253*sin(q1R))/4503599627370496))/36893488147419103232)))/36893488147419103232 - ((4503599440548691*cos(q4R))/4503599627370496 - (7514214926474921*sin(q4R))/36893488147419103232)*(cos(q3R)*(cos(q2R)*((2579692110316253*cos(q1R))/4503599627370496 - (1917820484151683*sin(q1R))/18014398509481984) - (32968958366167862000829996477285*sin(q2R))/40564819207303340847894502572032 + (7514214926474921*sin(q2R)*((1917820484151683*cos(q1R))/18014398509481984 + (2579692110316253*sin(q1R))/4503599627370496))/36893488147419103232) - (9007199067919185*sin(q3R)*((17274190877287359225804725738355*cos(q1R))/162259276829213363391578010288128 + (23235800371559029388956996013805*sin(q1R))/40564819207303340847894502572032 + 27504203825998033884751021716381/166153499473114484112975882535043072))/9007199254740992 + (7514214926474921*sin(q3R)*((32968958366167862000829996477285*cos(q2R))/40564819207303340847894502572032 - (7514214926474921*cos(q2R)*((1917820484151683*cos(q1R))/18014398509481984 + (2579692110316253*sin(q1R))/4503599627370496))/36893488147419103232 + sin(q2R)*((2579692110316253*cos(q1R))/4503599627370496 - (1917820484151683*sin(q1R))/18014398509481984)))/36893488147419103232) + ((234819211581865*cos(q4R))/1152921504606846976 + (9007199067919185*sin(q4R))/9007199254740992)*((129801982932889585091297864435361917839115294955*cos(q1R))/5986310706507378352962293074805895248510699696029696 + (296957971066013582975066703729047659005068212725*cos(q2R))/365375409332725729550921208179070754913983135744 + (174598797980560374072834504815488878557302284405*sin(q1R))/1496577676626844588240573268701473812127674924007424 - (67682029681889335677290557259385*cos(q2R)*((1917820484151683*cos(q1R))/18014398509481984 + (2579692110316253*sin(q1R))/4503599627370496))/332306998946228968225951765070086144 + (9007199067919185*sin(q2R)*((2579692110316253*cos(q1R))/4503599627370496 - (1917820484151683*sin(q1R))/18014398509481984))/9007199254740992 + 206672498930123057048696703425560088887371380901/6129982163463555433433388108601236734474956488734408704)))/36893488147419103232 + sin(q5R)*(((7514214926474921*cos(q4R))/36893488147419103232 + (4503599440548691*sin(q4R))/4503599627370496)*(cos(q3R)*(cos(q2R)*((2579692110316253*cos(q1R))/4503599627370496 - (1917820484151683*sin(q1R))/18014398509481984) - (32968958366167862000829996477285*sin(q2R))/40564819207303340847894502572032 + (7514214926474921*sin(q2R)*((1917820484151683*cos(q1R))/18014398509481984 + (2579692110316253*sin(q1R))/4503599627370496))/36893488147419103232) - (9007199067919185*sin(q3R)*((17274190877287359225804725738355*cos(q1R))/162259276829213363391578010288128 + (23235800371559029388956996013805*sin(q1R))/40564819207303340847894502572032 + 27504203825998033884751021716381/166153499473114484112975882535043072))/9007199254740992 + (7514214926474921*sin(q3R)*((32968958366167862000829996477285*cos(q2R))/40564819207303340847894502572032 - (7514214926474921*cos(q2R)*((1917820484151683*cos(q1R))/18014398509481984 + (2579692110316253*sin(q1R))/4503599627370496))/36893488147419103232 + sin(q2R)*((2579692110316253*cos(q1R))/4503599627370496 - (1917820484151683*sin(q1R))/18014398509481984)))/36893488147419103232) - (7514214926474921*sin(q4R)*((9007199067919185*cos(q3R)*((17274190877287359225804725738355*cos(q1R))/162259276829213363391578010288128 + (23235800371559029388956996013805*sin(q1R))/40564819207303340847894502572032 + 27504203825998033884751021716381/166153499473114484112975882535043072))/9007199254740992 - (7514214926474921*cos(q3R)*((32968958366167862000829996477285*cos(q2R))/40564819207303340847894502572032 - (7514214926474921*cos(q2R)*((1917820484151683*cos(q1R))/18014398509481984 + (2579692110316253*sin(q1R))/4503599627370496))/36893488147419103232 + sin(q2R)*((2579692110316253*cos(q1R))/4503599627370496 - (1917820484151683*sin(q1R))/18014398509481984)))/36893488147419103232 + sin(q3R)*(cos(q2R)*((2579692110316253*cos(q1R))/4503599627370496 - (1917820484151683*sin(q1R))/18014398509481984) - (32968958366167862000829996477285*sin(q2R))/40564819207303340847894502572032 + (7514214926474921*sin(q2R)*((1917820484151683*cos(q1R))/18014398509481984 + (2579692110316253*sin(q1R))/4503599627370496))/36893488147419103232)))/36893488147419103232 + ((9007199067919185*cos(q4R))/9007199254740992 - (234819211581865*sin(q4R))/1152921504606846976)*((129801982932889585091297864435361917839115294955*cos(q1R))/5986310706507378352962293074805895248510699696029696 + (296957971066013582975066703729047659005068212725*cos(q2R))/365375409332725729550921208179070754913983135744 + (174598797980560374072834504815488878557302284405*sin(q1R))/1496577676626844588240573268701473812127674924007424 - (67682029681889335677290557259385*cos(q2R)*((1917820484151683*cos(q1R))/18014398509481984 + (2579692110316253*sin(q1R))/4503599627370496))/332306998946228968225951765070086144 + (9007199067919185*sin(q2R)*((2579692110316253*cos(q1R))/4503599627370496 - (1917820484151683*sin(q1R))/18014398509481984))/9007199254740992 + 206672498930123057048696703425560088887371380901/6129982163463555433433388108601236734474956488734408704))))/332306998946228968225951765070086144000, 0; (584133382113593486367040631332731*sin(q6R)*((1528559695827542654859482295756575375660057523072748460051910118126597762297125*cos(q1R))/8343699359066055009355553539724812947666814540455674882605631280555545803830627148527195652096 + (3497003479222003021661409533057350838749300515155764632398442290070889008826875*cos(q2R))/509258994083621521567111422102344540262867098416484062659035112338595324940834176545849344 + (2056090974134078155817856050893176283501835309672875224633265471054954772650875*sin(q1R))/2085924839766513752338888384931203236916703635113918720651407820138886450957656787131798913024 - (609625514665592237562888769449172969868262801225*cos(q3R)*((17274190877287359225804725738355*cos(q1R))/162259276829213363391578010288128 + (23235800371559029388956996013805*sin(q1R))/40564819207303340847894502572032 + 27504203825998033884751021716381/166153499473114484112975882535043072))/2993155353253689176481146537402947624255349848014848 + (15893040848161638993908057577265778144967053025*sin(q3R)*((17274190877287359225804725738355*cos(q1R))/162259276829213363391578010288128 + (23235800371559029388956996013805*sin(q1R))/40564819207303340847894502572032 + 27504203825998033884751021716381/166153499473114484112975882535043072))/383123885216472214589586756787577295904684780545900544 - (9007199067919185*((4503599440548691*cos(q4R))/4503599627370496 - (7514214926474921*sin(q4R))/36893488147419103232)*(cos(q3R)*(cos(q2R)*((2579692110316253*cos(q1R))/4503599627370496 - (1917820484151683*sin(q1R))/18014398509481984) - (32968958366167862000829996477285*sin(q2R))/40564819207303340847894502572032 + (7514214926474921*sin(q2R)*((1917820484151683*cos(q1R))/18014398509481984 + (2579692110316253*sin(q1R))/4503599627370496))/36893488147419103232) - (9007199067919185*sin(q3R)*((17274190877287359225804725738355*cos(q1R))/162259276829213363391578010288128 + (23235800371559029388956996013805*sin(q1R))/40564819207303340847894502572032 + 27504203825998033884751021716381/166153499473114484112975882535043072))/9007199254740992 + (7514214926474921*sin(q3R)*((32968958366167862000829996477285*cos(q2R))/40564819207303340847894502572032 - (7514214926474921*cos(q2R)*((1917820484151683*cos(q1R))/18014398509481984 + (2579692110316253*sin(q1R))/4503599627370496))/36893488147419103232 + sin(q2R)*((2579692110316253*cos(q1R))/4503599627370496 - (1917820484151683*sin(q1R))/18014398509481984)))/36893488147419103232))/9007199254740992 + (508577317689771495245073589786522929324694383585*cos(q3R)*((32968958366167862000829996477285*cos(q2R))/40564819207303340847894502572032 - (7514214926474921*cos(q2R)*((1917820484151683*cos(q1R))/18014398509481984 + (2579692110316253*sin(q1R))/4503599627370496))/36893488147419103232 + sin(q2R)*((2579692110316253*cos(q1R))/4503599627370496 - (1917820484151683*sin(q1R))/18014398509481984)))/12259964326927110866866776217202473468949912977468817408 - (1764482024691522628700660907665*cos(q3R)*(cos(q2R)*((2579692110316253*cos(q1R))/4503599627370496 - (1917820484151683*sin(q1R))/18014398509481984) - (32968958366167862000829996477285*sin(q2R))/40564819207303340847894502572032 + (7514214926474921*sin(q2R)*((1917820484151683*cos(q1R))/18014398509481984 + (2579692110316253*sin(q1R))/4503599627370496))/36893488147419103232))/42535295865117307932921825928971026432 - (13258697167433729449897784796786197386719169465*sin(q3R)*((32968958366167862000829996477285*cos(q2R))/40564819207303340847894502572032 - (7514214926474921*cos(q2R)*((1917820484151683*cos(q1R))/18014398509481984 + (2579692110316253*sin(q1R))/4503599627370496))/36893488147419103232 + sin(q2R)*((2579692110316253*cos(q1R))/4503599627370496 - (1917820484151683*sin(q1R))/18014398509481984)))/1569275433846670190958947355801916604025588861116008628224 - (67682029681889335677290557259385*sin(q3R)*(cos(q2R)*((2579692110316253*cos(q1R))/4503599627370496 - (1917820484151683*sin(q1R))/18014398509481984) - (32968958366167862000829996477285*sin(q2R))/40564819207303340847894502572032 + (7514214926474921*sin(q2R)*((1917820484151683*cos(q1R))/18014398509481984 + (2579692110316253*sin(q1R))/4503599627370496))/36893488147419103232))/332306998946228968225951765070086144 + (67682029681889335677290557259385*cos(q4R)*((9007199067919185*cos(q3R)*((17274190877287359225804725738355*cos(q1R))/162259276829213363391578010288128 + (23235800371559029388956996013805*sin(q1R))/40564819207303340847894502572032 + 27504203825998033884751021716381/166153499473114484112975882535043072))/9007199254740992 - (7514214926474921*cos(q3R)*((32968958366167862000829996477285*cos(q2R))/40564819207303340847894502572032 - (7514214926474921*cos(q2R)*((1917820484151683*cos(q1R))/18014398509481984 + (2579692110316253*sin(q1R))/4503599627370496))/36893488147419103232 + sin(q2R)*((2579692110316253*cos(q1R))/4503599627370496 - (1917820484151683*sin(q1R))/18014398509481984)))/36893488147419103232 + sin(q3R)*(cos(q2R)*((2579692110316253*cos(q1R))/4503599627370496 - (1917820484151683*sin(q1R))/18014398509481984) - (32968958366167862000829996477285*sin(q2R))/40564819207303340847894502572032 + (7514214926474921*sin(q2R)*((1917820484151683*cos(q1R))/18014398509481984 + (2579692110316253*sin(q1R))/4503599627370496))/36893488147419103232)))/332306998946228968225951765070086144 + (9007199067919185*((234819211581865*cos(q4R))/1152921504606846976 + (9007199067919185*sin(q4R))/9007199254740992)*((129801982932889585091297864435361917839115294955*cos(q1R))/5986310706507378352962293074805895248510699696029696 + (296957971066013582975066703729047659005068212725*cos(q2R))/365375409332725729550921208179070754913983135744 + (174598797980560374072834504815488878557302284405*sin(q1R))/1496577676626844588240573268701473812127674924007424 - (67682029681889335677290557259385*cos(q2R)*((1917820484151683*cos(q1R))/18014398509481984 + (2579692110316253*sin(q1R))/4503599627370496))/332306998946228968225951765070086144 + (9007199067919185*sin(q2R)*((2579692110316253*cos(q1R))/4503599627370496 - (1917820484151683*sin(q1R))/18014398509481984))/9007199254740992 + 206672498930123057048696703425560088887371380901/6129982163463555433433388108601236734474956488734408704))/9007199254740992 - (797029601289130257223357069404502671534492977261568326111352375*cos(q2R)*((1917820484151683*cos(q1R))/18014398509481984 + (2579692110316253*sin(q1R))/4503599627370496))/463168356949264781694283940034751631413079938662562256157830336031652518559744 + (106069577339469832923929692356850887620017617375*sin(q2R)*((2579692110316253*cos(q1R))/4503599627370496 - (1917820484151683*sin(q1R))/18014398509481984))/12554203470773361527671578846415332832204710888928069025792 + 2433793729205816076131138531933890152433695130941136279164373721607455952153675/8543948143683640329580086824678208458410818089426611079788166431288878903122562200091848347746304))/16225927682921336339157801028812800 - (48638874966763599*cos(q6R)*((1528559695827542654859482295756575375660057523072748460051910118126597762297125*cos(q1R))/8343699359066055009355553539724812947666814540455674882605631280555545803830627148527195652096 + (3497003479222003021661409533057350838749300515155764632398442290070889008826875*cos(q2R))/509258994083621521567111422102344540262867098416484062659035112338595324940834176545849344 + (2056090974134078155817856050893176283501835309672875224633265471054954772650875*sin(q1R))/2085924839766513752338888384931203236916703635113918720651407820138886450957656787131798913024 - (609625514665592237562888769449172969868262801225*cos(q3R)*((17274190877287359225804725738355*cos(q1R))/162259276829213363391578010288128 + (23235800371559029388956996013805*sin(q1R))/40564819207303340847894502572032 + 27504203825998033884751021716381/166153499473114484112975882535043072))/2993155353253689176481146537402947624255349848014848 + (15893040848161638993908057577265778144967053025*sin(q3R)*((17274190877287359225804725738355*cos(q1R))/162259276829213363391578010288128 + (23235800371559029388956996013805*sin(q1R))/40564819207303340847894502572032 + 27504203825998033884751021716381/166153499473114484112975882535043072))/383123885216472214589586756787577295904684780545900544 - (9007199067919185*((4503599440548691*cos(q4R))/4503599627370496 - (7514214926474921*sin(q4R))/36893488147419103232)*(cos(q3R)*(cos(q2R)*((2579692110316253*cos(q1R))/4503599627370496 - (1917820484151683*sin(q1R))/18014398509481984) - (32968958366167862000829996477285*sin(q2R))/40564819207303340847894502572032 + (7514214926474921*sin(q2R)*((1917820484151683*cos(q1R))/18014398509481984 + (2579692110316253*sin(q1R))/4503599627370496))/36893488147419103232) - (9007199067919185*sin(q3R)*((17274190877287359225804725738355*cos(q1R))/162259276829213363391578010288128 + (23235800371559029388956996013805*sin(q1R))/40564819207303340847894502572032 + 27504203825998033884751021716381/166153499473114484112975882535043072))/9007199254740992 + (7514214926474921*sin(q3R)*((32968958366167862000829996477285*cos(q2R))/40564819207303340847894502572032 - (7514214926474921*cos(q2R)*((1917820484151683*cos(q1R))/18014398509481984 + (2579692110316253*sin(q1R))/4503599627370496))/36893488147419103232 + sin(q2R)*((2579692110316253*cos(q1R))/4503599627370496 - (1917820484151683*sin(q1R))/18014398509481984)))/36893488147419103232))/9007199254740992 + (508577317689771495245073589786522929324694383585*cos(q3R)*((32968958366167862000829996477285*cos(q2R))/40564819207303340847894502572032 - (7514214926474921*cos(q2R)*((1917820484151683*cos(q1R))/18014398509481984 + (2579692110316253*sin(q1R))/4503599627370496))/36893488147419103232 + sin(q2R)*((2579692110316253*cos(q1R))/4503599627370496 - (1917820484151683*sin(q1R))/18014398509481984)))/12259964326927110866866776217202473468949912977468817408 - (1764482024691522628700660907665*cos(q3R)*(cos(q2R)*((2579692110316253*cos(q1R))/4503599627370496 - (1917820484151683*sin(q1R))/18014398509481984) - (32968958366167862000829996477285*sin(q2R))/40564819207303340847894502572032 + (7514214926474921*sin(q2R)*((1917820484151683*cos(q1R))/18014398509481984 + (2579692110316253*sin(q1R))/4503599627370496))/36893488147419103232))/42535295865117307932921825928971026432 - (13258697167433729449897784796786197386719169465*sin(q3R)*((32968958366167862000829996477285*cos(q2R))/40564819207303340847894502572032 - (7514214926474921*cos(q2R)*((1917820484151683*cos(q1R))/18014398509481984 + (2579692110316253*sin(q1R))/4503599627370496))/36893488147419103232 + sin(q2R)*((2579692110316253*cos(q1R))/4503599627370496 - (1917820484151683*sin(q1R))/18014398509481984)))/1569275433846670190958947355801916604025588861116008628224 - (67682029681889335677290557259385*sin(q3R)*(cos(q2R)*((2579692110316253*cos(q1R))/4503599627370496 - (1917820484151683*sin(q1R))/18014398509481984) - (32968958366167862000829996477285*sin(q2R))/40564819207303340847894502572032 + (7514214926474921*sin(q2R)*((1917820484151683*cos(q1R))/18014398509481984 + (2579692110316253*sin(q1R))/4503599627370496))/36893488147419103232))/332306998946228968225951765070086144 + (67682029681889335677290557259385*cos(q4R)*((9007199067919185*cos(q3R)*((17274190877287359225804725738355*cos(q1R))/162259276829213363391578010288128 + (23235800371559029388956996013805*sin(q1R))/40564819207303340847894502572032 + 27504203825998033884751021716381/166153499473114484112975882535043072))/9007199254740992 - (7514214926474921*cos(q3R)*((32968958366167862000829996477285*cos(q2R))/40564819207303340847894502572032 - (7514214926474921*cos(q2R)*((1917820484151683*cos(q1R))/18014398509481984 + (2579692110316253*sin(q1R))/4503599627370496))/36893488147419103232 + sin(q2R)*((2579692110316253*cos(q1R))/4503599627370496 - (1917820484151683*sin(q1R))/18014398509481984)))/36893488147419103232 + sin(q3R)*(cos(q2R)*((2579692110316253*cos(q1R))/4503599627370496 - (1917820484151683*sin(q1R))/18014398509481984) - (32968958366167862000829996477285*sin(q2R))/40564819207303340847894502572032 + (7514214926474921*sin(q2R)*((1917820484151683*cos(q1R))/18014398509481984 + (2579692110316253*sin(q1R))/4503599627370496))/36893488147419103232)))/332306998946228968225951765070086144 + (9007199067919185*((234819211581865*cos(q4R))/1152921504606846976 + (9007199067919185*sin(q4R))/9007199254740992)*((129801982932889585091297864435361917839115294955*cos(q1R))/5986310706507378352962293074805895248510699696029696 + (296957971066013582975066703729047659005068212725*cos(q2R))/365375409332725729550921208179070754913983135744 + (174598797980560374072834504815488878557302284405*sin(q1R))/1496577676626844588240573268701473812127674924007424 - (67682029681889335677290557259385*cos(q2R)*((1917820484151683*cos(q1R))/18014398509481984 + (2579692110316253*sin(q1R))/4503599627370496))/332306998946228968225951765070086144 + (9007199067919185*sin(q2R)*((2579692110316253*cos(q1R))/4503599627370496 - (1917820484151683*sin(q1R))/18014398509481984))/9007199254740992 + 206672498930123057048696703425560088887371380901/6129982163463555433433388108601236734474956488734408704))/9007199254740992 - (797029601289130257223357069404502671534492977261568326111352375*cos(q2R)*((1917820484151683*cos(q1R))/18014398509481984 + (2579692110316253*sin(q1R))/4503599627370496))/463168356949264781694283940034751631413079938662562256157830336031652518559744 + (106069577339469832923929692356850887620017617375*sin(q2R)*((2579692110316253*cos(q1R))/4503599627370496 - (1917820484151683*sin(q1R))/18014398509481984))/12554203470773361527671578846415332832204710888928069025792 + 2433793729205816076131138531933890152433695130941136279164373721607455952153675/8543948143683640329580086824678208458410818089426611079788166431288878903122562200091848347746304))/1801439850948198400 - (27*sin(q6R)*(cos(q5R)*(((7514214926474921*cos(q4R))/36893488147419103232 + (4503599440548691*sin(q4R))/4503599627370496)*(cos(q3R)*(cos(q2R)*((2579692110316253*cos(q1R))/4503599627370496 - (1917820484151683*sin(q1R))/18014398509481984) - (32968958366167862000829996477285*sin(q2R))/40564819207303340847894502572032 + (7514214926474921*sin(q2R)*((1917820484151683*cos(q1R))/18014398509481984 + (2579692110316253*sin(q1R))/4503599627370496))/36893488147419103232) - (9007199067919185*sin(q3R)*((17274190877287359225804725738355*cos(q1R))/162259276829213363391578010288128 + (23235800371559029388956996013805*sin(q1R))/40564819207303340847894502572032 + 27504203825998033884751021716381/166153499473114484112975882535043072))/9007199254740992 + (7514214926474921*sin(q3R)*((32968958366167862000829996477285*cos(q2R))/40564819207303340847894502572032 - (7514214926474921*cos(q2R)*((1917820484151683*cos(q1R))/18014398509481984 + (2579692110316253*sin(q1R))/4503599627370496))/36893488147419103232 + sin(q2R)*((2579692110316253*cos(q1R))/4503599627370496 - (1917820484151683*sin(q1R))/18014398509481984)))/36893488147419103232) - (7514214926474921*sin(q4R)*((9007199067919185*cos(q3R)*((17274190877287359225804725738355*cos(q1R))/162259276829213363391578010288128 + (23235800371559029388956996013805*sin(q1R))/40564819207303340847894502572032 + 27504203825998033884751021716381/166153499473114484112975882535043072))/9007199254740992 - (7514214926474921*cos(q3R)*((32968958366167862000829996477285*cos(q2R))/40564819207303340847894502572032 - (7514214926474921*cos(q2R)*((1917820484151683*cos(q1R))/18014398509481984 + (2579692110316253*sin(q1R))/4503599627370496))/36893488147419103232 + sin(q2R)*((2579692110316253*cos(q1R))/4503599627370496 - (1917820484151683*sin(q1R))/18014398509481984)))/36893488147419103232 + sin(q3R)*(cos(q2R)*((2579692110316253*cos(q1R))/4503599627370496 - (1917820484151683*sin(q1R))/18014398509481984) - (32968958366167862000829996477285*sin(q2R))/40564819207303340847894502572032 + (7514214926474921*sin(q2R)*((1917820484151683*cos(q1R))/18014398509481984 + (2579692110316253*sin(q1R))/4503599627370496))/36893488147419103232)))/36893488147419103232 + ((9007199067919185*cos(q4R))/9007199254740992 - (234819211581865*sin(q4R))/1152921504606846976)*((129801982932889585091297864435361917839115294955*cos(q1R))/5986310706507378352962293074805895248510699696029696 + (296957971066013582975066703729047659005068212725*cos(q2R))/365375409332725729550921208179070754913983135744 + (174598797980560374072834504815488878557302284405*sin(q1R))/1496577676626844588240573268701473812127674924007424 - (67682029681889335677290557259385*cos(q2R)*((1917820484151683*cos(q1R))/18014398509481984 + (2579692110316253*sin(q1R))/4503599627370496))/332306998946228968225951765070086144 + (9007199067919185*sin(q2R)*((2579692110316253*cos(q1R))/4503599627370496 - (1917820484151683*sin(q1R))/18014398509481984))/9007199254740992 + 206672498930123057048696703425560088887371380901/6129982163463555433433388108601236734474956488734408704)) - (9007199067919185*sin(q5R)*((203422408166946418981152780445187297537016008229516441756292125*cos(q1R))/226156424291633194186662080095093570025917938800079226639565593765455331328 + (465385075279251052437186083221547446448384963368966483726351875*cos(q2R))/13803492693581127574869511724554050904902217944340773110325048447598592 + (273626851807209941619219010639387076236787289365779842797695875*sin(q1R))/56539106072908298546665520023773392506479484700019806659891398441363832832 - (81129635049124235038645691064225*cos(q3R)*((17274190877287359225804725738355*cos(q1R))/162259276829213363391578010288128 + (23235800371559029388956996013805*sin(q1R))/40564819207303340847894502572032 + 27504203825998033884751021716381/166153499473114484112975882535043072))/81129638414606681695789005144064 + (2115063383689692319117831580025*sin(q3R)*((17274190877287359225804725738355*cos(q1R))/162259276829213363391578010288128 + (23235800371559029388956996013805*sin(q1R))/40564819207303340847894502572032 + 27504203825998033884751021716381/166153499473114484112975882535043072))/10384593717069655257060992658440192 + (67682029681889335677290557259385*cos(q3R)*((32968958366167862000829996477285*cos(q2R))/40564819207303340847894502572032 - (7514214926474921*cos(q2R)*((1917820484151683*cos(q1R))/18014398509481984 + (2579692110316253*sin(q1R))/4503599627370496))/36893488147419103232 + sin(q2R)*((2579692110316253*cos(q1R))/4503599627370496 - (1917820484151683*sin(q1R))/18014398509481984)))/332306998946228968225951765070086144 - (234819211581865*cos(q3R)*(cos(q2R)*((2579692110316253*cos(q1R))/4503599627370496 - (1917820484151683*sin(q1R))/18014398509481984) - (32968958366167862000829996477285*sin(q2R))/40564819207303340847894502572032 + (7514214926474921*sin(q2R)*((1917820484151683*cos(q1R))/18014398509481984 + (2579692110316253*sin(q1R))/4503599627370496))/36893488147419103232))/1152921504606846976 - (1764482024691522628700660907665*sin(q3R)*((32968958366167862000829996477285*cos(q2R))/40564819207303340847894502572032 - (7514214926474921*cos(q2R)*((1917820484151683*cos(q1R))/18014398509481984 + (2579692110316253*sin(q1R))/4503599627370496))/36893488147419103232 + sin(q2R)*((2579692110316253*cos(q1R))/4503599627370496 - (1917820484151683*sin(q1R))/18014398509481984)))/42535295865117307932921825928971026432 - (9007199067919185*sin(q3R)*(cos(q2R)*((2579692110316253*cos(q1R))/4503599627370496 - (1917820484151683*sin(q1R))/18014398509481984) - (32968958366167862000829996477285*sin(q2R))/40564819207303340847894502572032 + (7514214926474921*sin(q2R)*((1917820484151683*cos(q1R))/18014398509481984 + (2579692110316253*sin(q1R))/4503599627370496))/36893488147419103232))/9007199254740992 - (106069577339469832923929692356850887620017617375*cos(q2R)*((1917820484151683*cos(q1R))/18014398509481984 + (2579692110316253*sin(q1R))/4503599627370496))/12554203470773361527671578846415332832204710888928069025792 + (14115856197532180673579726082375*sin(q2R)*((2579692110316253*cos(q1R))/4503599627370496 - (1917820484151683*sin(q1R))/18014398509481984))/340282366920938463463374607431768211456 + 323891950525769801103968238055131782751500431270071838086942675/231584178474632390847141970017375815706539969331281128078915168015826259279872))/9007199254740992 + (7514214926474921*sin(q5R)*((7514214926474921*cos(q4R)*((9007199067919185*cos(q3R)*((17274190877287359225804725738355*cos(q1R))/162259276829213363391578010288128 + (23235800371559029388956996013805*sin(q1R))/40564819207303340847894502572032 + 27504203825998033884751021716381/166153499473114484112975882535043072))/9007199254740992 - (7514214926474921*cos(q3R)*((32968958366167862000829996477285*cos(q2R))/40564819207303340847894502572032 - (7514214926474921*cos(q2R)*((1917820484151683*cos(q1R))/18014398509481984 + (2579692110316253*sin(q1R))/4503599627370496))/36893488147419103232 + sin(q2R)*((2579692110316253*cos(q1R))/4503599627370496 - (1917820484151683*sin(q1R))/18014398509481984)))/36893488147419103232 + sin(q3R)*(cos(q2R)*((2579692110316253*cos(q1R))/4503599627370496 - (1917820484151683*sin(q1R))/18014398509481984) - (32968958366167862000829996477285*sin(q2R))/40564819207303340847894502572032 + (7514214926474921*sin(q2R)*((1917820484151683*cos(q1R))/18014398509481984 + (2579692110316253*sin(q1R))/4503599627370496))/36893488147419103232)))/36893488147419103232 - ((4503599440548691*cos(q4R))/4503599627370496 - (7514214926474921*sin(q4R))/36893488147419103232)*(cos(q3R)*(cos(q2R)*((2579692110316253*cos(q1R))/4503599627370496 - (1917820484151683*sin(q1R))/18014398509481984) - (32968958366167862000829996477285*sin(q2R))/40564819207303340847894502572032 + (7514214926474921*sin(q2R)*((1917820484151683*cos(q1R))/18014398509481984 + (2579692110316253*sin(q1R))/4503599627370496))/36893488147419103232) - (9007199067919185*sin(q3R)*((17274190877287359225804725738355*cos(q1R))/162259276829213363391578010288128 + (23235800371559029388956996013805*sin(q1R))/40564819207303340847894502572032 + 27504203825998033884751021716381/166153499473114484112975882535043072))/9007199254740992 + (7514214926474921*sin(q3R)*((32968958366167862000829996477285*cos(q2R))/40564819207303340847894502572032 - (7514214926474921*cos(q2R)*((1917820484151683*cos(q1R))/18014398509481984 + (2579692110316253*sin(q1R))/4503599627370496))/36893488147419103232 + sin(q2R)*((2579692110316253*cos(q1R))/4503599627370496 - (1917820484151683*sin(q1R))/18014398509481984)))/36893488147419103232) + ((234819211581865*cos(q4R))/1152921504606846976 + (9007199067919185*sin(q4R))/9007199254740992)*((129801982932889585091297864435361917839115294955*cos(q1R))/5986310706507378352962293074805895248510699696029696 + (296957971066013582975066703729047659005068212725*cos(q2R))/365375409332725729550921208179070754913983135744 + (174598797980560374072834504815488878557302284405*sin(q1R))/1496577676626844588240573268701473812127674924007424 - (67682029681889335677290557259385*cos(q2R)*((1917820484151683*cos(q1R))/18014398509481984 + (2579692110316253*sin(q1R))/4503599627370496))/332306998946228968225951765070086144 + (9007199067919185*sin(q2R)*((2579692110316253*cos(q1R))/4503599627370496 - (1917820484151683*sin(q1R))/18014398509481984))/9007199254740992 + 206672498930123057048696703425560088887371380901/6129982163463555433433388108601236734474956488734408704)))/36893488147419103232))/1000 + (202883803014822867*cos(q6R)*((9007199067919185*cos(q5R)*((203422408166946418981152780445187297537016008229516441756292125*cos(q1R))/226156424291633194186662080095093570025917938800079226639565593765455331328 + (465385075279251052437186083221547446448384963368966483726351875*cos(q2R))/13803492693581127574869511724554050904902217944340773110325048447598592 + (273626851807209941619219010639387076236787289365779842797695875*sin(q1R))/56539106072908298546665520023773392506479484700019806659891398441363832832 - (81129635049124235038645691064225*cos(q3R)*((17274190877287359225804725738355*cos(q1R))/162259276829213363391578010288128 + (23235800371559029388956996013805*sin(q1R))/40564819207303340847894502572032 + 27504203825998033884751021716381/166153499473114484112975882535043072))/81129638414606681695789005144064 + (2115063383689692319117831580025*sin(q3R)*((17274190877287359225804725738355*cos(q1R))/162259276829213363391578010288128 + (23235800371559029388956996013805*sin(q1R))/40564819207303340847894502572032 + 27504203825998033884751021716381/166153499473114484112975882535043072))/10384593717069655257060992658440192 + (67682029681889335677290557259385*cos(q3R)*((32968958366167862000829996477285*cos(q2R))/40564819207303340847894502572032 - (7514214926474921*cos(q2R)*((1917820484151683*cos(q1R))/18014398509481984 + (2579692110316253*sin(q1R))/4503599627370496))/36893488147419103232 + sin(q2R)*((2579692110316253*cos(q1R))/4503599627370496 - (1917820484151683*sin(q1R))/18014398509481984)))/332306998946228968225951765070086144 - (234819211581865*cos(q3R)*(cos(q2R)*((2579692110316253*cos(q1R))/4503599627370496 - (1917820484151683*sin(q1R))/18014398509481984) - (32968958366167862000829996477285*sin(q2R))/40564819207303340847894502572032 + (7514214926474921*sin(q2R)*((1917820484151683*cos(q1R))/18014398509481984 + (2579692110316253*sin(q1R))/4503599627370496))/36893488147419103232))/1152921504606846976 - (1764482024691522628700660907665*sin(q3R)*((32968958366167862000829996477285*cos(q2R))/40564819207303340847894502572032 - (7514214926474921*cos(q2R)*((1917820484151683*cos(q1R))/18014398509481984 + (2579692110316253*sin(q1R))/4503599627370496))/36893488147419103232 + sin(q2R)*((2579692110316253*cos(q1R))/4503599627370496 - (1917820484151683*sin(q1R))/18014398509481984)))/42535295865117307932921825928971026432 - (9007199067919185*sin(q3R)*(cos(q2R)*((2579692110316253*cos(q1R))/4503599627370496 - (1917820484151683*sin(q1R))/18014398509481984) - (32968958366167862000829996477285*sin(q2R))/40564819207303340847894502572032 + (7514214926474921*sin(q2R)*((1917820484151683*cos(q1R))/18014398509481984 + (2579692110316253*sin(q1R))/4503599627370496))/36893488147419103232))/9007199254740992 - (106069577339469832923929692356850887620017617375*cos(q2R)*((1917820484151683*cos(q1R))/18014398509481984 + (2579692110316253*sin(q1R))/4503599627370496))/12554203470773361527671578846415332832204710888928069025792 + (14115856197532180673579726082375*sin(q2R)*((2579692110316253*cos(q1R))/4503599627370496 - (1917820484151683*sin(q1R))/18014398509481984))/340282366920938463463374607431768211456 + 323891950525769801103968238055131782751500431270071838086942675/231584178474632390847141970017375815706539969331281128078915168015826259279872))/9007199254740992 - (7514214926474921*cos(q5R)*((7514214926474921*cos(q4R)*((9007199067919185*cos(q3R)*((17274190877287359225804725738355*cos(q1R))/162259276829213363391578010288128 + (23235800371559029388956996013805*sin(q1R))/40564819207303340847894502572032 + 27504203825998033884751021716381/166153499473114484112975882535043072))/9007199254740992 - (7514214926474921*cos(q3R)*((32968958366167862000829996477285*cos(q2R))/40564819207303340847894502572032 - (7514214926474921*cos(q2R)*((1917820484151683*cos(q1R))/18014398509481984 + (2579692110316253*sin(q1R))/4503599627370496))/36893488147419103232 + sin(q2R)*((2579692110316253*cos(q1R))/4503599627370496 - (1917820484151683*sin(q1R))/18014398509481984)))/36893488147419103232 + sin(q3R)*(cos(q2R)*((2579692110316253*cos(q1R))/4503599627370496 - (1917820484151683*sin(q1R))/18014398509481984) - (32968958366167862000829996477285*sin(q2R))/40564819207303340847894502572032 + (7514214926474921*sin(q2R)*((1917820484151683*cos(q1R))/18014398509481984 + (2579692110316253*sin(q1R))/4503599627370496))/36893488147419103232)))/36893488147419103232 - ((4503599440548691*cos(q4R))/4503599627370496 - (7514214926474921*sin(q4R))/36893488147419103232)*(cos(q3R)*(cos(q2R)*((2579692110316253*cos(q1R))/4503599627370496 - (1917820484151683*sin(q1R))/18014398509481984) - (32968958366167862000829996477285*sin(q2R))/40564819207303340847894502572032 + (7514214926474921*sin(q2R)*((1917820484151683*cos(q1R))/18014398509481984 + (2579692110316253*sin(q1R))/4503599627370496))/36893488147419103232) - (9007199067919185*sin(q3R)*((17274190877287359225804725738355*cos(q1R))/162259276829213363391578010288128 + (23235800371559029388956996013805*sin(q1R))/40564819207303340847894502572032 + 27504203825998033884751021716381/166153499473114484112975882535043072))/9007199254740992 + (7514214926474921*sin(q3R)*((32968958366167862000829996477285*cos(q2R))/40564819207303340847894502572032 - (7514214926474921*cos(q2R)*((1917820484151683*cos(q1R))/18014398509481984 + (2579692110316253*sin(q1R))/4503599627370496))/36893488147419103232 + sin(q2R)*((2579692110316253*cos(q1R))/4503599627370496 - (1917820484151683*sin(q1R))/18014398509481984)))/36893488147419103232) + ((234819211581865*cos(q4R))/1152921504606846976 + (9007199067919185*sin(q4R))/9007199254740992)*((129801982932889585091297864435361917839115294955*cos(q1R))/5986310706507378352962293074805895248510699696029696 + (296957971066013582975066703729047659005068212725*cos(q2R))/365375409332725729550921208179070754913983135744 + (174598797980560374072834504815488878557302284405*sin(q1R))/1496577676626844588240573268701473812127674924007424 - (67682029681889335677290557259385*cos(q2R)*((1917820484151683*cos(q1R))/18014398509481984 + (2579692110316253*sin(q1R))/4503599627370496))/332306998946228968225951765070086144 + (9007199067919185*sin(q2R)*((2579692110316253*cos(q1R))/4503599627370496 - (1917820484151683*sin(q1R))/18014398509481984))/9007199254740992 + 206672498930123057048696703425560088887371380901/6129982163463555433433388108601236734474956488734408704)))/36893488147419103232 + sin(q5R)*(((7514214926474921*cos(q4R))/36893488147419103232 + (4503599440548691*sin(q4R))/4503599627370496)*(cos(q3R)*(cos(q2R)*((2579692110316253*cos(q1R))/4503599627370496 - (1917820484151683*sin(q1R))/18014398509481984) - (32968958366167862000829996477285*sin(q2R))/40564819207303340847894502572032 + (7514214926474921*sin(q2R)*((1917820484151683*cos(q1R))/18014398509481984 + (2579692110316253*sin(q1R))/4503599627370496))/36893488147419103232) - (9007199067919185*sin(q3R)*((17274190877287359225804725738355*cos(q1R))/162259276829213363391578010288128 + (23235800371559029388956996013805*sin(q1R))/40564819207303340847894502572032 + 27504203825998033884751021716381/166153499473114484112975882535043072))/9007199254740992 + (7514214926474921*sin(q3R)*((32968958366167862000829996477285*cos(q2R))/40564819207303340847894502572032 - (7514214926474921*cos(q2R)*((1917820484151683*cos(q1R))/18014398509481984 + (2579692110316253*sin(q1R))/4503599627370496))/36893488147419103232 + sin(q2R)*((2579692110316253*cos(q1R))/4503599627370496 - (1917820484151683*sin(q1R))/18014398509481984)))/36893488147419103232) - (7514214926474921*sin(q4R)*((9007199067919185*cos(q3R)*((17274190877287359225804725738355*cos(q1R))/162259276829213363391578010288128 + (23235800371559029388956996013805*sin(q1R))/40564819207303340847894502572032 + 27504203825998033884751021716381/166153499473114484112975882535043072))/9007199254740992 - (7514214926474921*cos(q3R)*((32968958366167862000829996477285*cos(q2R))/40564819207303340847894502572032 - (7514214926474921*cos(q2R)*((1917820484151683*cos(q1R))/18014398509481984 + (2579692110316253*sin(q1R))/4503599627370496))/36893488147419103232 + sin(q2R)*((2579692110316253*cos(q1R))/4503599627370496 - (1917820484151683*sin(q1R))/18014398509481984)))/36893488147419103232 + sin(q3R)*(cos(q2R)*((2579692110316253*cos(q1R))/4503599627370496 - (1917820484151683*sin(q1R))/18014398509481984) - (32968958366167862000829996477285*sin(q2R))/40564819207303340847894502572032 + (7514214926474921*sin(q2R)*((1917820484151683*cos(q1R))/18014398509481984 + (2579692110316253*sin(q1R))/4503599627370496))/36893488147419103232)))/36893488147419103232 + ((9007199067919185*cos(q4R))/9007199254740992 - (234819211581865*sin(q4R))/1152921504606846976)*((129801982932889585091297864435361917839115294955*cos(q1R))/5986310706507378352962293074805895248510699696029696 + (296957971066013582975066703729047659005068212725*cos(q2R))/365375409332725729550921208179070754913983135744 + (174598797980560374072834504815488878557302284405*sin(q1R))/1496577676626844588240573268701473812127674924007424 - (67682029681889335677290557259385*cos(q2R)*((1917820484151683*cos(q1R))/18014398509481984 + (2579692110316253*sin(q1R))/4503599627370496))/332306998946228968225951765070086144 + (9007199067919185*sin(q2R)*((2579692110316253*cos(q1R))/4503599627370496 - (1917820484151683*sin(q1R))/18014398509481984))/9007199254740992 + 206672498930123057048696703425560088887371380901/6129982163463555433433388108601236734474956488734408704))))/36893488147419103232000 - (324259171862923063*cos(q6R)*(cos(q5R)*(((7514214926474921*cos(q4R))/36893488147419103232 + (4503599440548691*sin(q4R))/4503599627370496)*(cos(q3R)*(cos(q2R)*((2579692110316253*cos(q1R))/4503599627370496 - (1917820484151683*sin(q1R))/18014398509481984) - (32968958366167862000829996477285*sin(q2R))/40564819207303340847894502572032 + (7514214926474921*sin(q2R)*((1917820484151683*cos(q1R))/18014398509481984 + (2579692110316253*sin(q1R))/4503599627370496))/36893488147419103232) - (9007199067919185*sin(q3R)*((17274190877287359225804725738355*cos(q1R))/162259276829213363391578010288128 + (23235800371559029388956996013805*sin(q1R))/40564819207303340847894502572032 + 27504203825998033884751021716381/166153499473114484112975882535043072))/9007199254740992 + (7514214926474921*sin(q3R)*((32968958366167862000829996477285*cos(q2R))/40564819207303340847894502572032 - (7514214926474921*cos(q2R)*((1917820484151683*cos(q1R))/18014398509481984 + (2579692110316253*sin(q1R))/4503599627370496))/36893488147419103232 + sin(q2R)*((2579692110316253*cos(q1R))/4503599627370496 - (1917820484151683*sin(q1R))/18014398509481984)))/36893488147419103232) - (7514214926474921*sin(q4R)*((9007199067919185*cos(q3R)*((17274190877287359225804725738355*cos(q1R))/162259276829213363391578010288128 + (23235800371559029388956996013805*sin(q1R))/40564819207303340847894502572032 + 27504203825998033884751021716381/166153499473114484112975882535043072))/9007199254740992 - (7514214926474921*cos(q3R)*((32968958366167862000829996477285*cos(q2R))/40564819207303340847894502572032 - (7514214926474921*cos(q2R)*((1917820484151683*cos(q1R))/18014398509481984 + (2579692110316253*sin(q1R))/4503599627370496))/36893488147419103232 + sin(q2R)*((2579692110316253*cos(q1R))/4503599627370496 - (1917820484151683*sin(q1R))/18014398509481984)))/36893488147419103232 + sin(q3R)*(cos(q2R)*((2579692110316253*cos(q1R))/4503599627370496 - (1917820484151683*sin(q1R))/18014398509481984) - (32968958366167862000829996477285*sin(q2R))/40564819207303340847894502572032 + (7514214926474921*sin(q2R)*((1917820484151683*cos(q1R))/18014398509481984 + (2579692110316253*sin(q1R))/4503599627370496))/36893488147419103232)))/36893488147419103232 + ((9007199067919185*cos(q4R))/9007199254740992 - (234819211581865*sin(q4R))/1152921504606846976)*((129801982932889585091297864435361917839115294955*cos(q1R))/5986310706507378352962293074805895248510699696029696 + (296957971066013582975066703729047659005068212725*cos(q2R))/365375409332725729550921208179070754913983135744 + (174598797980560374072834504815488878557302284405*sin(q1R))/1496577676626844588240573268701473812127674924007424 - (67682029681889335677290557259385*cos(q2R)*((1917820484151683*cos(q1R))/18014398509481984 + (2579692110316253*sin(q1R))/4503599627370496))/332306998946228968225951765070086144 + (9007199067919185*sin(q2R)*((2579692110316253*cos(q1R))/4503599627370496 - (1917820484151683*sin(q1R))/18014398509481984))/9007199254740992 + 206672498930123057048696703425560088887371380901/6129982163463555433433388108601236734474956488734408704)) - (9007199067919185*sin(q5R)*((203422408166946418981152780445187297537016008229516441756292125*cos(q1R))/226156424291633194186662080095093570025917938800079226639565593765455331328 + (465385075279251052437186083221547446448384963368966483726351875*cos(q2R))/13803492693581127574869511724554050904902217944340773110325048447598592 + (273626851807209941619219010639387076236787289365779842797695875*sin(q1R))/56539106072908298546665520023773392506479484700019806659891398441363832832 - (81129635049124235038645691064225*cos(q3R)*((17274190877287359225804725738355*cos(q1R))/162259276829213363391578010288128 + (23235800371559029388956996013805*sin(q1R))/40564819207303340847894502572032 + 27504203825998033884751021716381/166153499473114484112975882535043072))/81129638414606681695789005144064 + (2115063383689692319117831580025*sin(q3R)*((17274190877287359225804725738355*cos(q1R))/162259276829213363391578010288128 + (23235800371559029388956996013805*sin(q1R))/40564819207303340847894502572032 + 27504203825998033884751021716381/166153499473114484112975882535043072))/10384593717069655257060992658440192 + (67682029681889335677290557259385*cos(q3R)*((32968958366167862000829996477285*cos(q2R))/40564819207303340847894502572032 - (7514214926474921*cos(q2R)*((1917820484151683*cos(q1R))/18014398509481984 + (2579692110316253*sin(q1R))/4503599627370496))/36893488147419103232 + sin(q2R)*((2579692110316253*cos(q1R))/4503599627370496 - (1917820484151683*sin(q1R))/18014398509481984)))/332306998946228968225951765070086144 - (234819211581865*cos(q3R)*(cos(q2R)*((2579692110316253*cos(q1R))/4503599627370496 - (1917820484151683*sin(q1R))/18014398509481984) - (32968958366167862000829996477285*sin(q2R))/40564819207303340847894502572032 + (7514214926474921*sin(q2R)*((1917820484151683*cos(q1R))/18014398509481984 + (2579692110316253*sin(q1R))/4503599627370496))/36893488147419103232))/1152921504606846976 - (1764482024691522628700660907665*sin(q3R)*((32968958366167862000829996477285*cos(q2R))/40564819207303340847894502572032 - (7514214926474921*cos(q2R)*((1917820484151683*cos(q1R))/18014398509481984 + (2579692110316253*sin(q1R))/4503599627370496))/36893488147419103232 + sin(q2R)*((2579692110316253*cos(q1R))/4503599627370496 - (1917820484151683*sin(q1R))/18014398509481984)))/42535295865117307932921825928971026432 - (9007199067919185*sin(q3R)*(cos(q2R)*((2579692110316253*cos(q1R))/4503599627370496 - (1917820484151683*sin(q1R))/18014398509481984) - (32968958366167862000829996477285*sin(q2R))/40564819207303340847894502572032 + (7514214926474921*sin(q2R)*((1917820484151683*cos(q1R))/18014398509481984 + (2579692110316253*sin(q1R))/4503599627370496))/36893488147419103232))/9007199254740992 - (106069577339469832923929692356850887620017617375*cos(q2R)*((1917820484151683*cos(q1R))/18014398509481984 + (2579692110316253*sin(q1R))/4503599627370496))/12554203470773361527671578846415332832204710888928069025792 + (14115856197532180673579726082375*sin(q2R)*((2579692110316253*cos(q1R))/4503599627370496 - (1917820484151683*sin(q1R))/18014398509481984))/340282366920938463463374607431768211456 + 323891950525769801103968238055131782751500431270071838086942675/231584178474632390847141970017375815706539969331281128078915168015826259279872))/9007199254740992 + (7514214926474921*sin(q5R)*((7514214926474921*cos(q4R)*((9007199067919185*cos(q3R)*((17274190877287359225804725738355*cos(q1R))/162259276829213363391578010288128 + (23235800371559029388956996013805*sin(q1R))/40564819207303340847894502572032 + 27504203825998033884751021716381/166153499473114484112975882535043072))/9007199254740992 - (7514214926474921*cos(q3R)*((32968958366167862000829996477285*cos(q2R))/40564819207303340847894502572032 - (7514214926474921*cos(q2R)*((1917820484151683*cos(q1R))/18014398509481984 + (2579692110316253*sin(q1R))/4503599627370496))/36893488147419103232 + sin(q2R)*((2579692110316253*cos(q1R))/4503599627370496 - (1917820484151683*sin(q1R))/18014398509481984)))/36893488147419103232 + sin(q3R)*(cos(q2R)*((2579692110316253*cos(q1R))/4503599627370496 - (1917820484151683*sin(q1R))/18014398509481984) - (32968958366167862000829996477285*sin(q2R))/40564819207303340847894502572032 + (7514214926474921*sin(q2R)*((1917820484151683*cos(q1R))/18014398509481984 + (2579692110316253*sin(q1R))/4503599627370496))/36893488147419103232)))/36893488147419103232 - ((4503599440548691*cos(q4R))/4503599627370496 - (7514214926474921*sin(q4R))/36893488147419103232)*(cos(q3R)*(cos(q2R)*((2579692110316253*cos(q1R))/4503599627370496 - (1917820484151683*sin(q1R))/18014398509481984) - (32968958366167862000829996477285*sin(q2R))/40564819207303340847894502572032 + (7514214926474921*sin(q2R)*((1917820484151683*cos(q1R))/18014398509481984 + (2579692110316253*sin(q1R))/4503599627370496))/36893488147419103232) - (9007199067919185*sin(q3R)*((17274190877287359225804725738355*cos(q1R))/162259276829213363391578010288128 + (23235800371559029388956996013805*sin(q1R))/40564819207303340847894502572032 + 27504203825998033884751021716381/166153499473114484112975882535043072))/9007199254740992 + (7514214926474921*sin(q3R)*((32968958366167862000829996477285*cos(q2R))/40564819207303340847894502572032 - (7514214926474921*cos(q2R)*((1917820484151683*cos(q1R))/18014398509481984 + (2579692110316253*sin(q1R))/4503599627370496))/36893488147419103232 + sin(q2R)*((2579692110316253*cos(q1R))/4503599627370496 - (1917820484151683*sin(q1R))/18014398509481984)))/36893488147419103232) + ((234819211581865*cos(q4R))/1152921504606846976 + (9007199067919185*sin(q4R))/9007199254740992)*((129801982932889585091297864435361917839115294955*cos(q1R))/5986310706507378352962293074805895248510699696029696 + (296957971066013582975066703729047659005068212725*cos(q2R))/365375409332725729550921208179070754913983135744 + (174598797980560374072834504815488878557302284405*sin(q1R))/1496577676626844588240573268701473812127674924007424 - (67682029681889335677290557259385*cos(q2R)*((1917820484151683*cos(q1R))/18014398509481984 + (2579692110316253*sin(q1R))/4503599627370496))/332306998946228968225951765070086144 + (9007199067919185*sin(q2R)*((2579692110316253*cos(q1R))/4503599627370496 - (1917820484151683*sin(q1R))/18014398509481984))/9007199254740992 + 206672498930123057048696703425560088887371380901/6129982163463555433433388108601236734474956488734408704)))/36893488147419103232))/9007199254740992000 - (2436553109258773196144549622003023*sin(q6R)*((9007199067919185*cos(q5R)*((203422408166946418981152780445187297537016008229516441756292125*cos(q1R))/226156424291633194186662080095093570025917938800079226639565593765455331328 + (465385075279251052437186083221547446448384963368966483726351875*cos(q2R))/13803492693581127574869511724554050904902217944340773110325048447598592 + (273626851807209941619219010639387076236787289365779842797695875*sin(q1R))/56539106072908298546665520023773392506479484700019806659891398441363832832 - (81129635049124235038645691064225*cos(q3R)*((17274190877287359225804725738355*cos(q1R))/162259276829213363391578010288128 + (23235800371559029388956996013805*sin(q1R))/40564819207303340847894502572032 + 27504203825998033884751021716381/166153499473114484112975882535043072))/81129638414606681695789005144064 + (2115063383689692319117831580025*sin(q3R)*((17274190877287359225804725738355*cos(q1R))/162259276829213363391578010288128 + (23235800371559029388956996013805*sin(q1R))/40564819207303340847894502572032 + 27504203825998033884751021716381/166153499473114484112975882535043072))/10384593717069655257060992658440192 + (67682029681889335677290557259385*cos(q3R)*((32968958366167862000829996477285*cos(q2R))/40564819207303340847894502572032 - (7514214926474921*cos(q2R)*((1917820484151683*cos(q1R))/18014398509481984 + (2579692110316253*sin(q1R))/4503599627370496))/36893488147419103232 + sin(q2R)*((2579692110316253*cos(q1R))/4503599627370496 - (1917820484151683*sin(q1R))/18014398509481984)))/332306998946228968225951765070086144 - (234819211581865*cos(q3R)*(cos(q2R)*((2579692110316253*cos(q1R))/4503599627370496 - (1917820484151683*sin(q1R))/18014398509481984) - (32968958366167862000829996477285*sin(q2R))/40564819207303340847894502572032 + (7514214926474921*sin(q2R)*((1917820484151683*cos(q1R))/18014398509481984 + (2579692110316253*sin(q1R))/4503599627370496))/36893488147419103232))/1152921504606846976 - (1764482024691522628700660907665*sin(q3R)*((32968958366167862000829996477285*cos(q2R))/40564819207303340847894502572032 - (7514214926474921*cos(q2R)*((1917820484151683*cos(q1R))/18014398509481984 + (2579692110316253*sin(q1R))/4503599627370496))/36893488147419103232 + sin(q2R)*((2579692110316253*cos(q1R))/4503599627370496 - (1917820484151683*sin(q1R))/18014398509481984)))/42535295865117307932921825928971026432 - (9007199067919185*sin(q3R)*(cos(q2R)*((2579692110316253*cos(q1R))/4503599627370496 - (1917820484151683*sin(q1R))/18014398509481984) - (32968958366167862000829996477285*sin(q2R))/40564819207303340847894502572032 + (7514214926474921*sin(q2R)*((1917820484151683*cos(q1R))/18014398509481984 + (2579692110316253*sin(q1R))/4503599627370496))/36893488147419103232))/9007199254740992 - (106069577339469832923929692356850887620017617375*cos(q2R)*((1917820484151683*cos(q1R))/18014398509481984 + (2579692110316253*sin(q1R))/4503599627370496))/12554203470773361527671578846415332832204710888928069025792 + (14115856197532180673579726082375*sin(q2R)*((2579692110316253*cos(q1R))/4503599627370496 - (1917820484151683*sin(q1R))/18014398509481984))/340282366920938463463374607431768211456 + 323891950525769801103968238055131782751500431270071838086942675/231584178474632390847141970017375815706539969331281128078915168015826259279872))/9007199254740992 - (7514214926474921*cos(q5R)*((7514214926474921*cos(q4R)*((9007199067919185*cos(q3R)*((17274190877287359225804725738355*cos(q1R))/162259276829213363391578010288128 + (23235800371559029388956996013805*sin(q1R))/40564819207303340847894502572032 + 27504203825998033884751021716381/166153499473114484112975882535043072))/9007199254740992 - (7514214926474921*cos(q3R)*((32968958366167862000829996477285*cos(q2R))/40564819207303340847894502572032 - (7514214926474921*cos(q2R)*((1917820484151683*cos(q1R))/18014398509481984 + (2579692110316253*sin(q1R))/4503599627370496))/36893488147419103232 + sin(q2R)*((2579692110316253*cos(q1R))/4503599627370496 - (1917820484151683*sin(q1R))/18014398509481984)))/36893488147419103232 + sin(q3R)*(cos(q2R)*((2579692110316253*cos(q1R))/4503599627370496 - (1917820484151683*sin(q1R))/18014398509481984) - (32968958366167862000829996477285*sin(q2R))/40564819207303340847894502572032 + (7514214926474921*sin(q2R)*((1917820484151683*cos(q1R))/18014398509481984 + (2579692110316253*sin(q1R))/4503599627370496))/36893488147419103232)))/36893488147419103232 - ((4503599440548691*cos(q4R))/4503599627370496 - (7514214926474921*sin(q4R))/36893488147419103232)*(cos(q3R)*(cos(q2R)*((2579692110316253*cos(q1R))/4503599627370496 - (1917820484151683*sin(q1R))/18014398509481984) - (32968958366167862000829996477285*sin(q2R))/40564819207303340847894502572032 + (7514214926474921*sin(q2R)*((1917820484151683*cos(q1R))/18014398509481984 + (2579692110316253*sin(q1R))/4503599627370496))/36893488147419103232) - (9007199067919185*sin(q3R)*((17274190877287359225804725738355*cos(q1R))/162259276829213363391578010288128 + (23235800371559029388956996013805*sin(q1R))/40564819207303340847894502572032 + 27504203825998033884751021716381/166153499473114484112975882535043072))/9007199254740992 + (7514214926474921*sin(q3R)*((32968958366167862000829996477285*cos(q2R))/40564819207303340847894502572032 - (7514214926474921*cos(q2R)*((1917820484151683*cos(q1R))/18014398509481984 + (2579692110316253*sin(q1R))/4503599627370496))/36893488147419103232 + sin(q2R)*((2579692110316253*cos(q1R))/4503599627370496 - (1917820484151683*sin(q1R))/18014398509481984)))/36893488147419103232) + ((234819211581865*cos(q4R))/1152921504606846976 + (9007199067919185*sin(q4R))/9007199254740992)*((129801982932889585091297864435361917839115294955*cos(q1R))/5986310706507378352962293074805895248510699696029696 + (296957971066013582975066703729047659005068212725*cos(q2R))/365375409332725729550921208179070754913983135744 + (174598797980560374072834504815488878557302284405*sin(q1R))/1496577676626844588240573268701473812127674924007424 - (67682029681889335677290557259385*cos(q2R)*((1917820484151683*cos(q1R))/18014398509481984 + (2579692110316253*sin(q1R))/4503599627370496))/332306998946228968225951765070086144 + (9007199067919185*sin(q2R)*((2579692110316253*cos(q1R))/4503599627370496 - (1917820484151683*sin(q1R))/18014398509481984))/9007199254740992 + 206672498930123057048696703425560088887371380901/6129982163463555433433388108601236734474956488734408704)))/36893488147419103232 + sin(q5R)*(((7514214926474921*cos(q4R))/36893488147419103232 + (4503599440548691*sin(q4R))/4503599627370496)*(cos(q3R)*(cos(q2R)*((2579692110316253*cos(q1R))/4503599627370496 - (1917820484151683*sin(q1R))/18014398509481984) - (32968958366167862000829996477285*sin(q2R))/40564819207303340847894502572032 + (7514214926474921*sin(q2R)*((1917820484151683*cos(q1R))/18014398509481984 + (2579692110316253*sin(q1R))/4503599627370496))/36893488147419103232) - (9007199067919185*sin(q3R)*((17274190877287359225804725738355*cos(q1R))/162259276829213363391578010288128 + (23235800371559029388956996013805*sin(q1R))/40564819207303340847894502572032 + 27504203825998033884751021716381/166153499473114484112975882535043072))/9007199254740992 + (7514214926474921*sin(q3R)*((32968958366167862000829996477285*cos(q2R))/40564819207303340847894502572032 - (7514214926474921*cos(q2R)*((1917820484151683*cos(q1R))/18014398509481984 + (2579692110316253*sin(q1R))/4503599627370496))/36893488147419103232 + sin(q2R)*((2579692110316253*cos(q1R))/4503599627370496 - (1917820484151683*sin(q1R))/18014398509481984)))/36893488147419103232) - (7514214926474921*sin(q4R)*((9007199067919185*cos(q3R)*((17274190877287359225804725738355*cos(q1R))/162259276829213363391578010288128 + (23235800371559029388956996013805*sin(q1R))/40564819207303340847894502572032 + 27504203825998033884751021716381/166153499473114484112975882535043072))/9007199254740992 - (7514214926474921*cos(q3R)*((32968958366167862000829996477285*cos(q2R))/40564819207303340847894502572032 - (7514214926474921*cos(q2R)*((1917820484151683*cos(q1R))/18014398509481984 + (2579692110316253*sin(q1R))/4503599627370496))/36893488147419103232 + sin(q2R)*((2579692110316253*cos(q1R))/4503599627370496 - (1917820484151683*sin(q1R))/18014398509481984)))/36893488147419103232 + sin(q3R)*(cos(q2R)*((2579692110316253*cos(q1R))/4503599627370496 - (1917820484151683*sin(q1R))/18014398509481984) - (32968958366167862000829996477285*sin(q2R))/40564819207303340847894502572032 + (7514214926474921*sin(q2R)*((1917820484151683*cos(q1R))/18014398509481984 + (2579692110316253*sin(q1R))/4503599627370496))/36893488147419103232)))/36893488147419103232 + ((9007199067919185*cos(q4R))/9007199254740992 - (234819211581865*sin(q4R))/1152921504606846976)*((129801982932889585091297864435361917839115294955*cos(q1R))/5986310706507378352962293074805895248510699696029696 + (296957971066013582975066703729047659005068212725*cos(q2R))/365375409332725729550921208179070754913983135744 + (174598797980560374072834504815488878557302284405*sin(q1R))/1496577676626844588240573268701473812127674924007424 - (67682029681889335677290557259385*cos(q2R)*((1917820484151683*cos(q1R))/18014398509481984 + (2579692110316253*sin(q1R))/4503599627370496))/332306998946228968225951765070086144 + (9007199067919185*sin(q2R)*((2579692110316253*cos(q1R))/4503599627370496 - (1917820484151683*sin(q1R))/18014398509481984))/9007199254740992 + 206672498930123057048696703425560088887371380901/6129982163463555433433388108601236734474956488734408704))))/332306998946228968225951765070086144000, (2088071082526564406903398213797*cos(q2R))/202824096036516704239472512860160 + (74798728534121409375499805238398747969162575335180104128142834367071381686099963900677649745715814801813600055994310527932079337929*sin(q2R))/866459279412754643618254432544713657323886586054942679740774868942069158689258007199992001907543618155434753425438616196554424320000 + (81*((9007199067919185*cos(q4R))/9007199254740992 - (234819211581865*sin(q4R))/1152921504606846976)*((31346119847137124244279794758002175024246659075*sin(q2R))/91343852333181432387730302044767688728495783936 + (9007199067919185*cos(q2R)*((1392340654334763*cos(q1R))/2251799813685248 + (398031123528767*sin(q1R))/562949953421312))/9007199254740992 - (67682029681889335677290557259385*sin(q2R)*((398031123528767*cos(q1R))/562949953421312 - (1392340654334763*sin(q1R))/2251799813685248))/332306998946228968225951765070086144))/2000 - (81222263116692158804177042061221826384594597321566869716687*((234819211581865*cos(q4R))/1152921504606846976 + (9007199067919185*sin(q4R))/9007199254740992)*((31346119847137124244279794758002175024246659075*sin(q2R))/91343852333181432387730302044767688728495783936 + (9007199067919185*cos(q2R)*((1392340654334763*cos(q1R))/2251799813685248 + (398031123528767*sin(q1R))/562949953421312))/9007199254740992 - (67682029681889335677290557259385*sin(q2R)*((398031123528767*cos(q1R))/562949953421312 - (1392340654334763*sin(q1R))/2251799813685248))/332306998946228968225951765070086144))/306499108173177771671669405430061836723747824436720435200000 + (2436553109258773196144549622003023*cos(q6R)*(sin(q5R)*(((9007199067919185*cos(q4R))/9007199254740992 - (234819211581865*sin(q4R))/1152921504606846976)*((31346119847137124244279794758002175024246659075*sin(q2R))/91343852333181432387730302044767688728495783936 + (9007199067919185*cos(q2R)*((1392340654334763*cos(q1R))/2251799813685248 + (398031123528767*sin(q1R))/562949953421312))/9007199254740992 - (67682029681889335677290557259385*sin(q2R)*((398031123528767*cos(q1R))/562949953421312 - (1392340654334763*sin(q1R))/2251799813685248))/332306998946228968225951765070086144) + (7514214926474921*sin(q4R)*((7514214926474921*cos(q3R)*((3480118470877607344838997022995*sin(q2R))/10141204801825835211973625643008 + cos(q2R)*((1392340654334763*cos(q1R))/2251799813685248 + (398031123528767*sin(q1R))/562949953421312) - (7514214926474921*sin(q2R)*((398031123528767*cos(q1R))/562949953421312 - (1392340654334763*sin(q1R))/2251799813685248))/36893488147419103232))/36893488147419103232 + sin(q3R)*((7514214926474921*cos(q2R)*((398031123528767*cos(q1R))/562949953421312 - (1392340654334763*sin(q1R))/2251799813685248))/36893488147419103232 - (3480118470877607344838997022995*cos(q2R))/10141204801825835211973625643008 + sin(q2R)*((1392340654334763*cos(q1R))/2251799813685248 + (398031123528767*sin(q1R))/562949953421312))))/36893488147419103232 - ((7514214926474921*cos(q4R))/36893488147419103232 + (4503599440548691*sin(q4R))/4503599627370496)*(cos(q3R)*((7514214926474921*cos(q2R)*((398031123528767*cos(q1R))/562949953421312 - (1392340654334763*sin(q1R))/2251799813685248))/36893488147419103232 - (3480118470877607344838997022995*cos(q2R))/10141204801825835211973625643008 + sin(q2R)*((1392340654334763*cos(q1R))/2251799813685248 + (398031123528767*sin(q1R))/562949953421312)) - (7514214926474921*sin(q3R)*((3480118470877607344838997022995*sin(q2R))/10141204801825835211973625643008 + cos(q2R)*((1392340654334763*cos(q1R))/2251799813685248 + (398031123528767*sin(q1R))/562949953421312) - (7514214926474921*sin(q2R)*((398031123528767*cos(q1R))/562949953421312 - (1392340654334763*sin(q1R))/2251799813685248))/36893488147419103232))/36893488147419103232)) - (7514214926474921*cos(q5R)*(((234819211581865*cos(q4R))/1152921504606846976 + (9007199067919185*sin(q4R))/9007199254740992)*((31346119847137124244279794758002175024246659075*sin(q2R))/91343852333181432387730302044767688728495783936 + (9007199067919185*cos(q2R)*((1392340654334763*cos(q1R))/2251799813685248 + (398031123528767*sin(q1R))/562949953421312))/9007199254740992 - (67682029681889335677290557259385*sin(q2R)*((398031123528767*cos(q1R))/562949953421312 - (1392340654334763*sin(q1R))/2251799813685248))/332306998946228968225951765070086144) - (7514214926474921*cos(q4R)*((7514214926474921*cos(q3R)*((3480118470877607344838997022995*sin(q2R))/10141204801825835211973625643008 + cos(q2R)*((1392340654334763*cos(q1R))/2251799813685248 + (398031123528767*sin(q1R))/562949953421312) - (7514214926474921*sin(q2R)*((398031123528767*cos(q1R))/562949953421312 - (1392340654334763*sin(q1R))/2251799813685248))/36893488147419103232))/36893488147419103232 + sin(q3R)*((7514214926474921*cos(q2R)*((398031123528767*cos(q1R))/562949953421312 - (1392340654334763*sin(q1R))/2251799813685248))/36893488147419103232 - (3480118470877607344838997022995*cos(q2R))/10141204801825835211973625643008 + sin(q2R)*((1392340654334763*cos(q1R))/2251799813685248 + (398031123528767*sin(q1R))/562949953421312))))/36893488147419103232 + ((4503599440548691*cos(q4R))/4503599627370496 - (7514214926474921*sin(q4R))/36893488147419103232)*(cos(q3R)*((7514214926474921*cos(q2R)*((398031123528767*cos(q1R))/562949953421312 - (1392340654334763*sin(q1R))/2251799813685248))/36893488147419103232 - (3480118470877607344838997022995*cos(q2R))/10141204801825835211973625643008 + sin(q2R)*((1392340654334763*cos(q1R))/2251799813685248 + (398031123528767*sin(q1R))/562949953421312)) - (7514214926474921*sin(q3R)*((3480118470877607344838997022995*sin(q2R))/10141204801825835211973625643008 + cos(q2R)*((1392340654334763*cos(q1R))/2251799813685248 + (398031123528767*sin(q1R))/562949953421312) - (7514214926474921*sin(q2R)*((398031123528767*cos(q1R))/562949953421312 - (1392340654334763*sin(q1R))/2251799813685248))/36893488147419103232))/36893488147419103232)))/36893488147419103232 + (9007199067919185*cos(q5R)*((49124851885283889459147163519037433596494512994900179139213125*sin(q2R))/3450873173395281893717377931138512726225554486085193277581262111899648 + (234819211581865*cos(q3R)*((7514214926474921*cos(q2R)*((398031123528767*cos(q1R))/562949953421312 - (1392340654334763*sin(q1R))/2251799813685248))/36893488147419103232 - (3480118470877607344838997022995*cos(q2R))/10141204801825835211973625643008 + sin(q2R)*((1392340654334763*cos(q1R))/2251799813685248 + (398031123528767*sin(q1R))/562949953421312)))/1152921504606846976 + (67682029681889335677290557259385*cos(q3R)*((3480118470877607344838997022995*sin(q2R))/10141204801825835211973625643008 + cos(q2R)*((1392340654334763*cos(q1R))/2251799813685248 + (398031123528767*sin(q1R))/562949953421312) - (7514214926474921*sin(q2R)*((398031123528767*cos(q1R))/562949953421312 - (1392340654334763*sin(q1R))/2251799813685248))/36893488147419103232))/332306998946228968225951765070086144 + (9007199067919185*sin(q3R)*((7514214926474921*cos(q2R)*((398031123528767*cos(q1R))/562949953421312 - (1392340654334763*sin(q1R))/2251799813685248))/36893488147419103232 - (3480118470877607344838997022995*cos(q2R))/10141204801825835211973625643008 + sin(q2R)*((1392340654334763*cos(q1R))/2251799813685248 + (398031123528767*sin(q1R))/562949953421312)))/9007199254740992 - (1764482024691522628700660907665*sin(q3R)*((3480118470877607344838997022995*sin(q2R))/10141204801825835211973625643008 + cos(q2R)*((1392340654334763*cos(q1R))/2251799813685248 + (398031123528767*sin(q1R))/562949953421312) - (7514214926474921*sin(q2R)*((398031123528767*cos(q1R))/562949953421312 - (1392340654334763*sin(q1R))/2251799813685248))/36893488147419103232))/42535295865117307932921825928971026432 + (14115856197532180673579726082375*cos(q2R)*((1392340654334763*cos(q1R))/2251799813685248 + (398031123528767*sin(q1R))/562949953421312))/340282366920938463463374607431768211456 - (106069577339469832923929692356850887620017617375*sin(q2R)*((398031123528767*cos(q1R))/562949953421312 - (1392340654334763*sin(q1R))/2251799813685248))/12554203470773361527671578846415332832204710888928069025792))/9007199254740992))/332306998946228968225951765070086144000 - (60617164743372705924380750591060836759586313939367162716784907429017787816377231*cos(q3R)*((7514214926474921*cos(q2R)*((398031123528767*cos(q1R))/562949953421312 - (1392340654334763*sin(q1R))/2251799813685248))/36893488147419103232 - (3480118470877607344838997022995*cos(q2R))/10141204801825835211973625643008 + sin(q2R)*((1392340654334763*cos(q1R))/2251799813685248 + (398031123528767*sin(q1R))/562949953421312)))/1447401115466452442794637312608598848165874808320507050493219800098914120499200000 + (27*cos(q6R)*((7514214926474921*sin(q5R)*(((234819211581865*cos(q4R))/1152921504606846976 + (9007199067919185*sin(q4R))/9007199254740992)*((31346119847137124244279794758002175024246659075*sin(q2R))/91343852333181432387730302044767688728495783936 + (9007199067919185*cos(q2R)*((1392340654334763*cos(q1R))/2251799813685248 + (398031123528767*sin(q1R))/562949953421312))/9007199254740992 - (67682029681889335677290557259385*sin(q2R)*((398031123528767*cos(q1R))/562949953421312 - (1392340654334763*sin(q1R))/2251799813685248))/332306998946228968225951765070086144) - (7514214926474921*cos(q4R)*((7514214926474921*cos(q3R)*((3480118470877607344838997022995*sin(q2R))/10141204801825835211973625643008 + cos(q2R)*((1392340654334763*cos(q1R))/2251799813685248 + (398031123528767*sin(q1R))/562949953421312) - (7514214926474921*sin(q2R)*((398031123528767*cos(q1R))/562949953421312 - (1392340654334763*sin(q1R))/2251799813685248))/36893488147419103232))/36893488147419103232 + sin(q3R)*((7514214926474921*cos(q2R)*((398031123528767*cos(q1R))/562949953421312 - (1392340654334763*sin(q1R))/2251799813685248))/36893488147419103232 - (3480118470877607344838997022995*cos(q2R))/10141204801825835211973625643008 + sin(q2R)*((1392340654334763*cos(q1R))/2251799813685248 + (398031123528767*sin(q1R))/562949953421312))))/36893488147419103232 + ((4503599440548691*cos(q4R))/4503599627370496 - (7514214926474921*sin(q4R))/36893488147419103232)*(cos(q3R)*((7514214926474921*cos(q2R)*((398031123528767*cos(q1R))/562949953421312 - (1392340654334763*sin(q1R))/2251799813685248))/36893488147419103232 - (3480118470877607344838997022995*cos(q2R))/10141204801825835211973625643008 + sin(q2R)*((1392340654334763*cos(q1R))/2251799813685248 + (398031123528767*sin(q1R))/562949953421312)) - (7514214926474921*sin(q3R)*((3480118470877607344838997022995*sin(q2R))/10141204801825835211973625643008 + cos(q2R)*((1392340654334763*cos(q1R))/2251799813685248 + (398031123528767*sin(q1R))/562949953421312) - (7514214926474921*sin(q2R)*((398031123528767*cos(q1R))/562949953421312 - (1392340654334763*sin(q1R))/2251799813685248))/36893488147419103232))/36893488147419103232)))/36893488147419103232 + cos(q5R)*(((9007199067919185*cos(q4R))/9007199254740992 - (234819211581865*sin(q4R))/1152921504606846976)*((31346119847137124244279794758002175024246659075*sin(q2R))/91343852333181432387730302044767688728495783936 + (9007199067919185*cos(q2R)*((1392340654334763*cos(q1R))/2251799813685248 + (398031123528767*sin(q1R))/562949953421312))/9007199254740992 - (67682029681889335677290557259385*sin(q2R)*((398031123528767*cos(q1R))/562949953421312 - (1392340654334763*sin(q1R))/2251799813685248))/332306998946228968225951765070086144) + (7514214926474921*sin(q4R)*((7514214926474921*cos(q3R)*((3480118470877607344838997022995*sin(q2R))/10141204801825835211973625643008 + cos(q2R)*((1392340654334763*cos(q1R))/2251799813685248 + (398031123528767*sin(q1R))/562949953421312) - (7514214926474921*sin(q2R)*((398031123528767*cos(q1R))/562949953421312 - (1392340654334763*sin(q1R))/2251799813685248))/36893488147419103232))/36893488147419103232 + sin(q3R)*((7514214926474921*cos(q2R)*((398031123528767*cos(q1R))/562949953421312 - (1392340654334763*sin(q1R))/2251799813685248))/36893488147419103232 - (3480118470877607344838997022995*cos(q2R))/10141204801825835211973625643008 + sin(q2R)*((1392340654334763*cos(q1R))/2251799813685248 + (398031123528767*sin(q1R))/562949953421312))))/36893488147419103232 - ((7514214926474921*cos(q4R))/36893488147419103232 + (4503599440548691*sin(q4R))/4503599627370496)*(cos(q3R)*((7514214926474921*cos(q2R)*((398031123528767*cos(q1R))/562949953421312 - (1392340654334763*sin(q1R))/2251799813685248))/36893488147419103232 - (3480118470877607344838997022995*cos(q2R))/10141204801825835211973625643008 + sin(q2R)*((1392340654334763*cos(q1R))/2251799813685248 + (398031123528767*sin(q1R))/562949953421312)) - (7514214926474921*sin(q3R)*((3480118470877607344838997022995*sin(q2R))/10141204801825835211973625643008 + cos(q2R)*((1392340654334763*cos(q1R))/2251799813685248 + (398031123528767*sin(q1R))/562949953421312) - (7514214926474921*sin(q2R)*((398031123528767*cos(q1R))/562949953421312 - (1392340654334763*sin(q1R))/2251799813685248))/36893488147419103232))/36893488147419103232)) - (9007199067919185*sin(q5R)*((49124851885283889459147163519037433596494512994900179139213125*sin(q2R))/3450873173395281893717377931138512726225554486085193277581262111899648 + (234819211581865*cos(q3R)*((7514214926474921*cos(q2R)*((398031123528767*cos(q1R))/562949953421312 - (1392340654334763*sin(q1R))/2251799813685248))/36893488147419103232 - (3480118470877607344838997022995*cos(q2R))/10141204801825835211973625643008 + sin(q2R)*((1392340654334763*cos(q1R))/2251799813685248 + (398031123528767*sin(q1R))/562949953421312)))/1152921504606846976 + (67682029681889335677290557259385*cos(q3R)*((3480118470877607344838997022995*sin(q2R))/10141204801825835211973625643008 + cos(q2R)*((1392340654334763*cos(q1R))/2251799813685248 + (398031123528767*sin(q1R))/562949953421312) - (7514214926474921*sin(q2R)*((398031123528767*cos(q1R))/562949953421312 - (1392340654334763*sin(q1R))/2251799813685248))/36893488147419103232))/332306998946228968225951765070086144 + (9007199067919185*sin(q3R)*((7514214926474921*cos(q2R)*((398031123528767*cos(q1R))/562949953421312 - (1392340654334763*sin(q1R))/2251799813685248))/36893488147419103232 - (3480118470877607344838997022995*cos(q2R))/10141204801825835211973625643008 + sin(q2R)*((1392340654334763*cos(q1R))/2251799813685248 + (398031123528767*sin(q1R))/562949953421312)))/9007199254740992 - (1764482024691522628700660907665*sin(q3R)*((3480118470877607344838997022995*sin(q2R))/10141204801825835211973625643008 + cos(q2R)*((1392340654334763*cos(q1R))/2251799813685248 + (398031123528767*sin(q1R))/562949953421312) - (7514214926474921*sin(q2R)*((398031123528767*cos(q1R))/562949953421312 - (1392340654334763*sin(q1R))/2251799813685248))/36893488147419103232))/42535295865117307932921825928971026432 + (14115856197532180673579726082375*cos(q2R)*((1392340654334763*cos(q1R))/2251799813685248 + (398031123528767*sin(q1R))/562949953421312))/340282366920938463463374607431768211456 - (106069577339469832923929692356850887620017617375*sin(q2R)*((398031123528767*cos(q1R))/562949953421312 - (1392340654334763*sin(q1R))/2251799813685248))/12554203470773361527671578846415332832204710888928069025792))/9007199254740992))/1000 + (202883803014822867*sin(q6R)*(sin(q5R)*(((9007199067919185*cos(q4R))/9007199254740992 - (234819211581865*sin(q4R))/1152921504606846976)*((31346119847137124244279794758002175024246659075*sin(q2R))/91343852333181432387730302044767688728495783936 + (9007199067919185*cos(q2R)*((1392340654334763*cos(q1R))/2251799813685248 + (398031123528767*sin(q1R))/562949953421312))/9007199254740992 - (67682029681889335677290557259385*sin(q2R)*((398031123528767*cos(q1R))/562949953421312 - (1392340654334763*sin(q1R))/2251799813685248))/332306998946228968225951765070086144) + (7514214926474921*sin(q4R)*((7514214926474921*cos(q3R)*((3480118470877607344838997022995*sin(q2R))/10141204801825835211973625643008 + cos(q2R)*((1392340654334763*cos(q1R))/2251799813685248 + (398031123528767*sin(q1R))/562949953421312) - (7514214926474921*sin(q2R)*((398031123528767*cos(q1R))/562949953421312 - (1392340654334763*sin(q1R))/2251799813685248))/36893488147419103232))/36893488147419103232 + sin(q3R)*((7514214926474921*cos(q2R)*((398031123528767*cos(q1R))/562949953421312 - (1392340654334763*sin(q1R))/2251799813685248))/36893488147419103232 - (3480118470877607344838997022995*cos(q2R))/10141204801825835211973625643008 + sin(q2R)*((1392340654334763*cos(q1R))/2251799813685248 + (398031123528767*sin(q1R))/562949953421312))))/36893488147419103232 - ((7514214926474921*cos(q4R))/36893488147419103232 + (4503599440548691*sin(q4R))/4503599627370496)*(cos(q3R)*((7514214926474921*cos(q2R)*((398031123528767*cos(q1R))/562949953421312 - (1392340654334763*sin(q1R))/2251799813685248))/36893488147419103232 - (3480118470877607344838997022995*cos(q2R))/10141204801825835211973625643008 + sin(q2R)*((1392340654334763*cos(q1R))/2251799813685248 + (398031123528767*sin(q1R))/562949953421312)) - (7514214926474921*sin(q3R)*((3480118470877607344838997022995*sin(q2R))/10141204801825835211973625643008 + cos(q2R)*((1392340654334763*cos(q1R))/2251799813685248 + (398031123528767*sin(q1R))/562949953421312) - (7514214926474921*sin(q2R)*((398031123528767*cos(q1R))/562949953421312 - (1392340654334763*sin(q1R))/2251799813685248))/36893488147419103232))/36893488147419103232)) - (7514214926474921*cos(q5R)*(((234819211581865*cos(q4R))/1152921504606846976 + (9007199067919185*sin(q4R))/9007199254740992)*((31346119847137124244279794758002175024246659075*sin(q2R))/91343852333181432387730302044767688728495783936 + (9007199067919185*cos(q2R)*((1392340654334763*cos(q1R))/2251799813685248 + (398031123528767*sin(q1R))/562949953421312))/9007199254740992 - (67682029681889335677290557259385*sin(q2R)*((398031123528767*cos(q1R))/562949953421312 - (1392340654334763*sin(q1R))/2251799813685248))/332306998946228968225951765070086144) - (7514214926474921*cos(q4R)*((7514214926474921*cos(q3R)*((3480118470877607344838997022995*sin(q2R))/10141204801825835211973625643008 + cos(q2R)*((1392340654334763*cos(q1R))/2251799813685248 + (398031123528767*sin(q1R))/562949953421312) - (7514214926474921*sin(q2R)*((398031123528767*cos(q1R))/562949953421312 - (1392340654334763*sin(q1R))/2251799813685248))/36893488147419103232))/36893488147419103232 + sin(q3R)*((7514214926474921*cos(q2R)*((398031123528767*cos(q1R))/562949953421312 - (1392340654334763*sin(q1R))/2251799813685248))/36893488147419103232 - (3480118470877607344838997022995*cos(q2R))/10141204801825835211973625643008 + sin(q2R)*((1392340654334763*cos(q1R))/2251799813685248 + (398031123528767*sin(q1R))/562949953421312))))/36893488147419103232 + ((4503599440548691*cos(q4R))/4503599627370496 - (7514214926474921*sin(q4R))/36893488147419103232)*(cos(q3R)*((7514214926474921*cos(q2R)*((398031123528767*cos(q1R))/562949953421312 - (1392340654334763*sin(q1R))/2251799813685248))/36893488147419103232 - (3480118470877607344838997022995*cos(q2R))/10141204801825835211973625643008 + sin(q2R)*((1392340654334763*cos(q1R))/2251799813685248 + (398031123528767*sin(q1R))/562949953421312)) - (7514214926474921*sin(q3R)*((3480118470877607344838997022995*sin(q2R))/10141204801825835211973625643008 + cos(q2R)*((1392340654334763*cos(q1R))/2251799813685248 + (398031123528767*sin(q1R))/562949953421312) - (7514214926474921*sin(q2R)*((398031123528767*cos(q1R))/562949953421312 - (1392340654334763*sin(q1R))/2251799813685248))/36893488147419103232))/36893488147419103232)))/36893488147419103232 + (9007199067919185*cos(q5R)*((49124851885283889459147163519037433596494512994900179139213125*sin(q2R))/3450873173395281893717377931138512726225554486085193277581262111899648 + (234819211581865*cos(q3R)*((7514214926474921*cos(q2R)*((398031123528767*cos(q1R))/562949953421312 - (1392340654334763*sin(q1R))/2251799813685248))/36893488147419103232 - (3480118470877607344838997022995*cos(q2R))/10141204801825835211973625643008 + sin(q2R)*((1392340654334763*cos(q1R))/2251799813685248 + (398031123528767*sin(q1R))/562949953421312)))/1152921504606846976 + (67682029681889335677290557259385*cos(q3R)*((3480118470877607344838997022995*sin(q2R))/10141204801825835211973625643008 + cos(q2R)*((1392340654334763*cos(q1R))/2251799813685248 + (398031123528767*sin(q1R))/562949953421312) - (7514214926474921*sin(q2R)*((398031123528767*cos(q1R))/562949953421312 - (1392340654334763*sin(q1R))/2251799813685248))/36893488147419103232))/332306998946228968225951765070086144 + (9007199067919185*sin(q3R)*((7514214926474921*cos(q2R)*((398031123528767*cos(q1R))/562949953421312 - (1392340654334763*sin(q1R))/2251799813685248))/36893488147419103232 - (3480118470877607344838997022995*cos(q2R))/10141204801825835211973625643008 + sin(q2R)*((1392340654334763*cos(q1R))/2251799813685248 + (398031123528767*sin(q1R))/562949953421312)))/9007199254740992 - (1764482024691522628700660907665*sin(q3R)*((3480118470877607344838997022995*sin(q2R))/10141204801825835211973625643008 + cos(q2R)*((1392340654334763*cos(q1R))/2251799813685248 + (398031123528767*sin(q1R))/562949953421312) - (7514214926474921*sin(q2R)*((398031123528767*cos(q1R))/562949953421312 - (1392340654334763*sin(q1R))/2251799813685248))/36893488147419103232))/42535295865117307932921825928971026432 + (14115856197532180673579726082375*cos(q2R)*((1392340654334763*cos(q1R))/2251799813685248 + (398031123528767*sin(q1R))/562949953421312))/340282366920938463463374607431768211456 - (106069577339469832923929692356850887620017617375*sin(q2R)*((398031123528767*cos(q1R))/562949953421312 - (1392340654334763*sin(q1R))/2251799813685248))/12554203470773361527671578846415332832204710888928069025792))/9007199254740992))/36893488147419103232000 - (347469655025336708709976918716104493695816557877713443586884917071777956519687017125887603*cos(q3R)*((3480118470877607344838997022995*sin(q2R))/10141204801825835211973625643008 + cos(q2R)*((1392340654334763*cos(q1R))/2251799813685248 + (398031123528767*sin(q1R))/562949953421312) - (7514214926474921*sin(q2R)*((398031123528767*cos(q1R))/562949953421312 - (1392340654334763*sin(q1R))/2251799813685248))/36893488147419103232))/83436993590660550093555535397248129476668145404556748826056312805555458038306271485271956520960000 - (46241644459901303158631016767207157814229090534989303509431886332469146043*sin(q3R)*((7514214926474921*cos(q2R)*((398031123528767*cos(q1R))/562949953421312 - (1392340654334763*sin(q1R))/2251799813685248))/36893488147419103232 - (3480118470877607344838997022995*cos(q2R))/10141204801825835211973625643008 + sin(q2R)*((1392340654334763*cos(q1R))/2251799813685248 + (398031123528767*sin(q1R))/562949953421312)))/2261564242916331941866620800950935700259179388000792266395655937654553313280000 - (324259171862923063*sin(q6R)*((7514214926474921*sin(q5R)*(((234819211581865*cos(q4R))/1152921504606846976 + (9007199067919185*sin(q4R))/9007199254740992)*((31346119847137124244279794758002175024246659075*sin(q2R))/91343852333181432387730302044767688728495783936 + (9007199067919185*cos(q2R)*((1392340654334763*cos(q1R))/2251799813685248 + (398031123528767*sin(q1R))/562949953421312))/9007199254740992 - (67682029681889335677290557259385*sin(q2R)*((398031123528767*cos(q1R))/562949953421312 - (1392340654334763*sin(q1R))/2251799813685248))/332306998946228968225951765070086144) - (7514214926474921*cos(q4R)*((7514214926474921*cos(q3R)*((3480118470877607344838997022995*sin(q2R))/10141204801825835211973625643008 + cos(q2R)*((1392340654334763*cos(q1R))/2251799813685248 + (398031123528767*sin(q1R))/562949953421312) - (7514214926474921*sin(q2R)*((398031123528767*cos(q1R))/562949953421312 - (1392340654334763*sin(q1R))/2251799813685248))/36893488147419103232))/36893488147419103232 + sin(q3R)*((7514214926474921*cos(q2R)*((398031123528767*cos(q1R))/562949953421312 - (1392340654334763*sin(q1R))/2251799813685248))/36893488147419103232 - (3480118470877607344838997022995*cos(q2R))/10141204801825835211973625643008 + sin(q2R)*((1392340654334763*cos(q1R))/2251799813685248 + (398031123528767*sin(q1R))/562949953421312))))/36893488147419103232 + ((4503599440548691*cos(q4R))/4503599627370496 - (7514214926474921*sin(q4R))/36893488147419103232)*(cos(q3R)*((7514214926474921*cos(q2R)*((398031123528767*cos(q1R))/562949953421312 - (1392340654334763*sin(q1R))/2251799813685248))/36893488147419103232 - (3480118470877607344838997022995*cos(q2R))/10141204801825835211973625643008 + sin(q2R)*((1392340654334763*cos(q1R))/2251799813685248 + (398031123528767*sin(q1R))/562949953421312)) - (7514214926474921*sin(q3R)*((3480118470877607344838997022995*sin(q2R))/10141204801825835211973625643008 + cos(q2R)*((1392340654334763*cos(q1R))/2251799813685248 + (398031123528767*sin(q1R))/562949953421312) - (7514214926474921*sin(q2R)*((398031123528767*cos(q1R))/562949953421312 - (1392340654334763*sin(q1R))/2251799813685248))/36893488147419103232))/36893488147419103232)))/36893488147419103232 + cos(q5R)*(((9007199067919185*cos(q4R))/9007199254740992 - (234819211581865*sin(q4R))/1152921504606846976)*((31346119847137124244279794758002175024246659075*sin(q2R))/91343852333181432387730302044767688728495783936 + (9007199067919185*cos(q2R)*((1392340654334763*cos(q1R))/2251799813685248 + (398031123528767*sin(q1R))/562949953421312))/9007199254740992 - (67682029681889335677290557259385*sin(q2R)*((398031123528767*cos(q1R))/562949953421312 - (1392340654334763*sin(q1R))/2251799813685248))/332306998946228968225951765070086144) + (7514214926474921*sin(q4R)*((7514214926474921*cos(q3R)*((3480118470877607344838997022995*sin(q2R))/10141204801825835211973625643008 + cos(q2R)*((1392340654334763*cos(q1R))/2251799813685248 + (398031123528767*sin(q1R))/562949953421312) - (7514214926474921*sin(q2R)*((398031123528767*cos(q1R))/562949953421312 - (1392340654334763*sin(q1R))/2251799813685248))/36893488147419103232))/36893488147419103232 + sin(q3R)*((7514214926474921*cos(q2R)*((398031123528767*cos(q1R))/562949953421312 - (1392340654334763*sin(q1R))/2251799813685248))/36893488147419103232 - (3480118470877607344838997022995*cos(q2R))/10141204801825835211973625643008 + sin(q2R)*((1392340654334763*cos(q1R))/2251799813685248 + (398031123528767*sin(q1R))/562949953421312))))/36893488147419103232 - ((7514214926474921*cos(q4R))/36893488147419103232 + (4503599440548691*sin(q4R))/4503599627370496)*(cos(q3R)*((7514214926474921*cos(q2R)*((398031123528767*cos(q1R))/562949953421312 - (1392340654334763*sin(q1R))/2251799813685248))/36893488147419103232 - (3480118470877607344838997022995*cos(q2R))/10141204801825835211973625643008 + sin(q2R)*((1392340654334763*cos(q1R))/2251799813685248 + (398031123528767*sin(q1R))/562949953421312)) - (7514214926474921*sin(q3R)*((3480118470877607344838997022995*sin(q2R))/10141204801825835211973625643008 + cos(q2R)*((1392340654334763*cos(q1R))/2251799813685248 + (398031123528767*sin(q1R))/562949953421312) - (7514214926474921*sin(q2R)*((398031123528767*cos(q1R))/562949953421312 - (1392340654334763*sin(q1R))/2251799813685248))/36893488147419103232))/36893488147419103232)) - (9007199067919185*sin(q5R)*((49124851885283889459147163519037433596494512994900179139213125*sin(q2R))/3450873173395281893717377931138512726225554486085193277581262111899648 + (234819211581865*cos(q3R)*((7514214926474921*cos(q2R)*((398031123528767*cos(q1R))/562949953421312 - (1392340654334763*sin(q1R))/2251799813685248))/36893488147419103232 - (3480118470877607344838997022995*cos(q2R))/10141204801825835211973625643008 + sin(q2R)*((1392340654334763*cos(q1R))/2251799813685248 + (398031123528767*sin(q1R))/562949953421312)))/1152921504606846976 + (67682029681889335677290557259385*cos(q3R)*((3480118470877607344838997022995*sin(q2R))/10141204801825835211973625643008 + cos(q2R)*((1392340654334763*cos(q1R))/2251799813685248 + (398031123528767*sin(q1R))/562949953421312) - (7514214926474921*sin(q2R)*((398031123528767*cos(q1R))/562949953421312 - (1392340654334763*sin(q1R))/2251799813685248))/36893488147419103232))/332306998946228968225951765070086144 + (9007199067919185*sin(q3R)*((7514214926474921*cos(q2R)*((398031123528767*cos(q1R))/562949953421312 - (1392340654334763*sin(q1R))/2251799813685248))/36893488147419103232 - (3480118470877607344838997022995*cos(q2R))/10141204801825835211973625643008 + sin(q2R)*((1392340654334763*cos(q1R))/2251799813685248 + (398031123528767*sin(q1R))/562949953421312)))/9007199254740992 - (1764482024691522628700660907665*sin(q3R)*((3480118470877607344838997022995*sin(q2R))/10141204801825835211973625643008 + cos(q2R)*((1392340654334763*cos(q1R))/2251799813685248 + (398031123528767*sin(q1R))/562949953421312) - (7514214926474921*sin(q2R)*((398031123528767*cos(q1R))/562949953421312 - (1392340654334763*sin(q1R))/2251799813685248))/36893488147419103232))/42535295865117307932921825928971026432 + (14115856197532180673579726082375*cos(q2R)*((1392340654334763*cos(q1R))/2251799813685248 + (398031123528767*sin(q1R))/562949953421312))/340282366920938463463374607431768211456 - (106069577339469832923929692356850887620017617375*sin(q2R)*((398031123528767*cos(q1R))/562949953421312 - (1392340654334763*sin(q1R))/2251799813685248))/12554203470773361527671578846415332832204710888928069025792))/9007199254740992))/9007199254740992000 + (455490404115240510935077772268745492204390157443214084883134054419271951750419293234291596923751*sin(q3R)*((3480118470877607344838997022995*sin(q2R))/10141204801825835211973625643008 + cos(q2R)*((1392340654334763*cos(q1R))/2251799813685248 + (398031123528767*sin(q1R))/562949953421312) - (7514214926474921*sin(q2R)*((398031123528767*cos(q1R))/562949953421312 - (1392340654334763*sin(q1R))/2251799813685248))/36893488147419103232))/53399675898022752059875542654238802865067613058916319248676040195555493144516013750574052173414400000 - (584133382113593486367040631332731*cos(q6R)*((369134695297269865703468593411141398729137707824460658574000083747077986538125*sin(q2R))/127314748520905380391777855525586135065716774604121015664758778084648831235208544136462336 + (9007199067919185*((234819211581865*cos(q4R))/1152921504606846976 + (9007199067919185*sin(q4R))/9007199254740992)*((31346119847137124244279794758002175024246659075*sin(q2R))/91343852333181432387730302044767688728495783936 + (9007199067919185*cos(q2R)*((1392340654334763*cos(q1R))/2251799813685248 + (398031123528767*sin(q1R))/562949953421312))/9007199254740992 - (67682029681889335677290557259385*sin(q2R)*((398031123528767*cos(q1R))/562949953421312 - (1392340654334763*sin(q1R))/2251799813685248))/332306998946228968225951765070086144))/9007199254740992 + (1764482024691522628700660907665*cos(q3R)*((7514214926474921*cos(q2R)*((398031123528767*cos(q1R))/562949953421312 - (1392340654334763*sin(q1R))/2251799813685248))/36893488147419103232 - (3480118470877607344838997022995*cos(q2R))/10141204801825835211973625643008 + sin(q2R)*((1392340654334763*cos(q1R))/2251799813685248 + (398031123528767*sin(q1R))/562949953421312)))/42535295865117307932921825928971026432 + (508577317689771495245073589786522929324694383585*cos(q3R)*((3480118470877607344838997022995*sin(q2R))/10141204801825835211973625643008 + cos(q2R)*((1392340654334763*cos(q1R))/2251799813685248 + (398031123528767*sin(q1R))/562949953421312) - (7514214926474921*sin(q2R)*((398031123528767*cos(q1R))/562949953421312 - (1392340654334763*sin(q1R))/2251799813685248))/36893488147419103232))/12259964326927110866866776217202473468949912977468817408 + (67682029681889335677290557259385*sin(q3R)*((7514214926474921*cos(q2R)*((398031123528767*cos(q1R))/562949953421312 - (1392340654334763*sin(q1R))/2251799813685248))/36893488147419103232 - (3480118470877607344838997022995*cos(q2R))/10141204801825835211973625643008 + sin(q2R)*((1392340654334763*cos(q1R))/2251799813685248 + (398031123528767*sin(q1R))/562949953421312)))/332306998946228968225951765070086144 - (13258697167433729449897784796786197386719169465*sin(q3R)*((3480118470877607344838997022995*sin(q2R))/10141204801825835211973625643008 + cos(q2R)*((1392340654334763*cos(q1R))/2251799813685248 + (398031123528767*sin(q1R))/562949953421312) - (7514214926474921*sin(q2R)*((398031123528767*cos(q1R))/562949953421312 - (1392340654334763*sin(q1R))/2251799813685248))/36893488147419103232))/1569275433846670190958947355801916604025588861116008628224 + (106069577339469832923929692356850887620017617375*cos(q2R)*((1392340654334763*cos(q1R))/2251799813685248 + (398031123528767*sin(q1R))/562949953421312))/12554203470773361527671578846415332832204710888928069025792 - (797029601289130257223357069404502671534492977261568326111352375*sin(q2R)*((398031123528767*cos(q1R))/562949953421312 - (1392340654334763*sin(q1R))/2251799813685248))/463168356949264781694283940034751631413079938662562256157830336031652518559744 - (67682029681889335677290557259385*cos(q4R)*((7514214926474921*cos(q3R)*((3480118470877607344838997022995*sin(q2R))/10141204801825835211973625643008 + cos(q2R)*((1392340654334763*cos(q1R))/2251799813685248 + (398031123528767*sin(q1R))/562949953421312) - (7514214926474921*sin(q2R)*((398031123528767*cos(q1R))/562949953421312 - (1392340654334763*sin(q1R))/2251799813685248))/36893488147419103232))/36893488147419103232 + sin(q3R)*((7514214926474921*cos(q2R)*((398031123528767*cos(q1R))/562949953421312 - (1392340654334763*sin(q1R))/2251799813685248))/36893488147419103232 - (3480118470877607344838997022995*cos(q2R))/10141204801825835211973625643008 + sin(q2R)*((1392340654334763*cos(q1R))/2251799813685248 + (398031123528767*sin(q1R))/562949953421312))))/332306998946228968225951765070086144 + (9007199067919185*((4503599440548691*cos(q4R))/4503599627370496 - 